simulink model "HVDCMMCInterconnection"  (R2023b)
settings: Solver=FixedStepDiscrete  StartTime=0.0  StopTime=10  FixedStep=Ts_Power  RelTol=1e-4
PreLoadFcn:
  | HVDCMMCInterconnectionParam
StartFcn:
  | tic
StopFcn:
  | toc
values from neighbouring files (symbols this model uses):
  C_PM = 1.758e-3    (= 0.001758)    [HVDCMMCInterconnectionParam.m]
  Cg = 50e-9    (= 5e-08)    [HVDCMMCInterconnectionParam.m]
  D_R = 0.001    [HVDCMMCInterconnectionParam.m]
  D_Rs = 1e8    (= 100000000)    [HVDCMMCInterconnectionParam.m]
  D_Vf = 0    [HVDCMMCInterconnectionParam.m]
  Fnom = 50    [HVDCMMCInterconnectionParam.m]
  HRM = 2    [HVDCMMCInterconnectionParam.m]
  Ki_Ireg = 6    [HVDCMMCInterconnectionParam.m]
  Ki_Preg = 1.0    (= 1)    [HVDCMMCInterconnectionParam.m]
  Ki_Qreg = 1.0    (= 1)    [HVDCMMCInterconnectionParam.m]
  Ki_VDCreg = 100    [HVDCMMCInterconnectionParam.m]
  Kp_Ireg = 0.6    [HVDCMMCInterconnectionParam.m]
  Kp_Preg = 0.5/3    (= 0.166666666667)    [HVDCMMCInterconnectionParam.m]
  Kp_Qreg = 0.5/3    (= 0.166666666667)    [HVDCMMCInterconnectionParam.m]
  Kp_VDCreg = 4    [HVDCMMCInterconnectionParam.m]
  L_cable = 15e-3    (= 0.015)    [HVDCMMCInterconnectionParam.m]
  Larm = Larm_pu*(Zb_ac/(2*pi*Fnom))    [HVDCMMCInterconnectionParam.m]
  Lff = Larm_pu/2    (= 0.075)    [HVDCMMCInterconnectionParam.m]
  Limits_Ireg = [ 2.0  -2.0]    [HVDCMMCInterconnectionParam.m]
  Limits_Preg = [ 1.2, 0.8 ]    [HVDCMMCInterconnectionParam.m]
  Limits_Qreg = [ 0.25, -0.25 ]    [HVDCMMCInterconnectionParam.m]
  Limits_VDCreg = [ 2.0  -2.0]    [HVDCMMCInterconnectionParam.m]
  Lxfo = 0.12    [HVDCMMCInterconnectionParam.m]
  Nb_PM = 36    [HVDCMMCInterconnectionParam.m]
  Pnom = 1000e6    (= 1000000000)    [HVDCMMCInterconnectionParam.m]
  R_cable = 0.5    [HVDCMMCInterconnectionParam.m]
  R_startup = 400    [HVDCMMCInterconnectionParam.m]
  Rarm = Rarm_pu*Zb_ac    [HVDCMMCInterconnectionParam.m]
  Rff = Rarm_pu/2    (= 0.00075)    [HVDCMMCInterconnectionParam.m]
  Rg = 100    [HVDCMMCInterconnectionParam.m]
  Rxfo = 0.003    [HVDCMMCInterconnectionParam.m]
  Slope_Pref = 0.5    [HVDCMMCInterconnectionParam.m]
  Slope_Qref = 0.5    [HVDCMMCInterconnectionParam.m]
  Slope_Vdc_ref = Vnom_dc/5    (= 128000)    [HVDCMMCInterconnectionParam.m]
  Tbrk1_On = 0.1    [HVDCMMCInterconnectionParam.m]
  Tbrk2_On = 1.0    (= 1)    [HVDCMMCInterconnectionParam.m]
  Tdeblock = 1.5    [HVDCMMCInterconnectionParam.m]
  Tfault = 9999    [HVDCMMCInterconnectionParam.m]
  Ton_Converter2 = 4    [HVDCMMCInterconnectionParam.m]
  Ton_PQreg = 4    [HVDCMMCInterconnectionParam.m]
  Ton_VDCreg = 1.5    [HVDCMMCInterconnectionParam.m]
  Ts = Ts_Control    (= 4e-05)    [HVDCMMCInterconnectionParam.m]    (also in power_circ2ss_sps_calc.m = 1e-06)
  Ts_Control = 40e-6    (= 4e-05)    [HVDCMMCInterconnectionParam.m]
  Ts_Power = 20e-6    (= 2e-05)    [HVDCMMCInterconnectionParam.m]
  Vb_ac = sqrt(2/3)*Vnom_sec    [HVDCMMCInterconnectionParam.m]
  Vb_dc = Vnom_dc    (= 640000)    [HVDCMMCInterconnectionParam.m]
  Vc0_PM = 0    [HVDCMMCInterconnectionParam.m]
  Vnom_dc = 640e3    (= 640000)    [HVDCMMCInterconnectionParam.m]
  Vnom_prim = 400e3    (= 400000)    [HVDCMMCInterconnectionParam.m]
  Vnom_sec = 333e3    (= 333000)    [HVDCMMCInterconnectionParam.m]
  w = 2*pi*Fnom    (= 314.159265359)    [HVDCMMCInterconnectionParam.m]
undefined symbols (not defined in the file or in its folder): ACDC, ACDC3, DiscIntNeverNeededParam, gcbh, Pcc, S, sps_AC, sps_rtmsupport
libraries: simulink x61, spsControlledVoltageSourceLib x56, spsCurrentMeasurementLib x56, spsDiodeLib x40, spsSeriesRLCBranchLib x32, spsVoltageMeasurementLib x20, powerlib_extras x9, spsHalfBridgeMMCmodel x8, spsGroundLib x7, spsSecondOrderFilterLib x6, spsabctodq0Lib x6, spsMeanLib x3
(part 1 of 11)
settings Model: SimulationMode=accelerator  Creator=The MathWorks, Inc.  LastModifiedBy=rober
settings SolverCC: ZeroCrossAlgorithm=Adaptive  InsertRTBMode=Always
settings DataIOCC: SaveFormat=StructureWithTime  SaveOutput=off  SignalLogging=off  DSMLogging=off  SaveTime=off  ReturnWorkspaceOutputs=off
settings OptimizationCC: ReuseModelBlockBuffer=off  ExpressionDepthLimit=2147483647  LifeSpan=inf
settings DebuggingCC: UnderspecifiedInitializationDetection=Classic  MergeDetectMultiDrivingBlocksExec=none  SolverPrmCheckMsg=warning  FcnCallInpInsideContextMsg=warning  AllowSymbolicDim=off  StateNameClashWarn=warning  SFUnexpectedBacktrackingDiag=warning  SFNoUnconditionalDefaultTransitionDiag=warning  SFExecutionAtInitializationDiag=none  ArithmeticOperatorsInVariantConditions=warning
settings HardwareCC: ProdBitPerPointer=32  ProdBitPerSizeT=32  ProdBitPerPtrDiffT=32  ProdLargestAtomicFloat=None  ProdIntDivRoundTo=Undefined  ProdEndianess=Unspecified  ProdWordSize=32  ProdHWDeviceType=32-bit Generic
settings ModelReferenceCC: EnableRefExpFcnMdlSchedulingChecks=on  EnableParallelModelReferenceBuilds=on  ModelReferenceMinAlgLoopOccurrences=on  PropagateSignalLabelsOutOfModel=off
settings SFSimCC: SimUseLocalCustomCode=off  CustomCodeUndefinedFunction=UseInterfaceOnly
settings RTWCC: RTWUseLocalCustomCode=off
settings CodeAppCC: StateflowObjectComments=on
settings GRTTargetCC: CombineOutputUpdateFcns=off  GRTInterface=on
settings ConfigComp: CovMetricSettings=dw  CovSaveCumulativeToWorkspaceVar=on  CovSaveSingleToWorkspaceVar=on  CovExternalEMLEnable=off
settings SimscapeCC: SimscapeNormalizeSystem=off

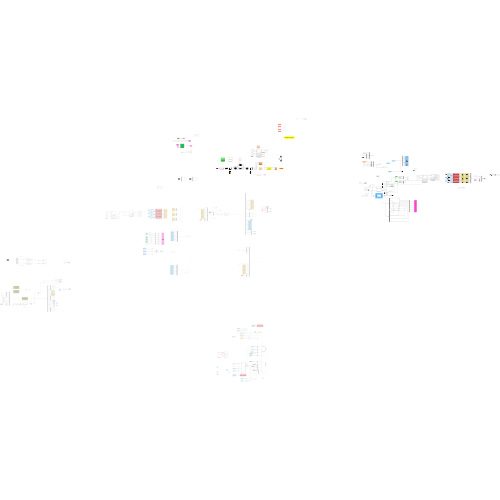
[thumbnail: Simulink's stored preview of the top-level diagram]
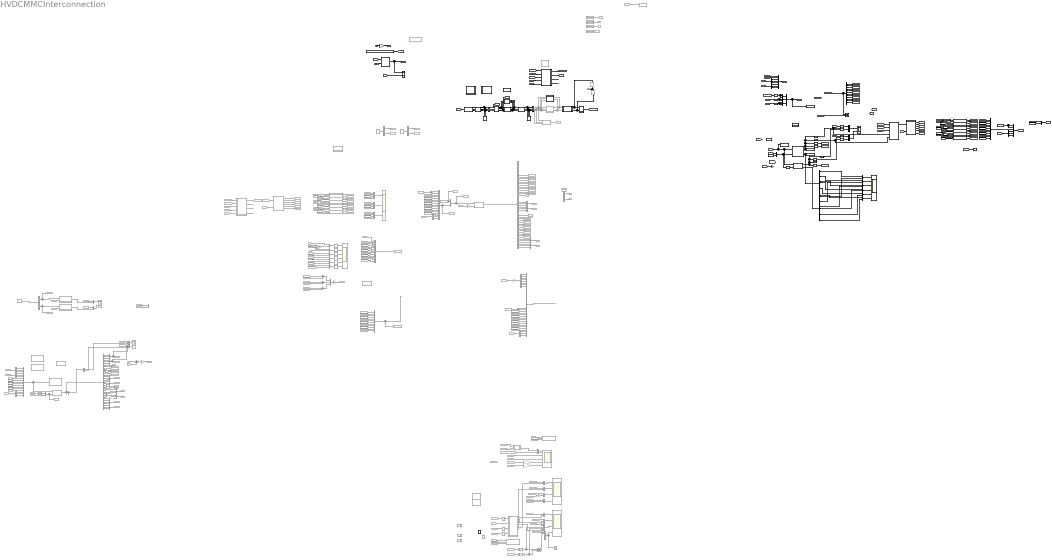
== system HVDCMMCInterconnection ==
  note: HVDC-MMC Control System
  3ph SM1 : Subsystem  Commented=on
  3ph SM10 : Subsystem
  3ph SM11 : Subsystem
  3ph SM12 : Subsystem
  3ph SM13 : Subsystem
  3ph SM14 : Subsystem
  3ph SM2 : Subsystem  Commented=on
  3ph SM3 : Subsystem  Commented=on
  3ph SM4 : Subsystem  Commented=on
  3ph SM5 : Subsystem  Commented=on
  3ph SM6 : Subsystem  Commented=on
  3ph SM7 : Subsystem  Commented=on
  3ph SM8 : Subsystem  Commented=on
  3ph SM9 : Subsystem
  Add1 : Sum  Commented=on  Inputs=-+
  BRK_CTRL : Subsystem  Commented=on
  BRK_CTRL1 : Subsystem  Commented=on
  Brk1 : spsThreePhaseBreakerLib/Three-Phase Breaker  InitialState=open  SwitchA=on  SwitchB=on  SwitchC=on  SwitchTimes=0.1  External=on  BreakerResistance=0.01  SnubberResistance=1e6  SnubberCapacitance=inf  Measurements=None
  Brk2 : spsThreePhaseBreakerLib/Three-Phase Breaker  InitialState=open  SwitchA=on  SwitchB=on  SwitchC=on  SwitchTimes=[30/60]*10000  External=on  BreakerResistance=0.01  SnubberResistance=1e6  SnubberCapacitance=inf  Measurements=None
  COMPARE1 : Scope  Commented=on  NumInputPorts=6
  COMPARE2 : Scope  NumInputPorts=6
  Cast To Double : DataTypeConversion  Commented=on  OutDataTypeStr=double  SaturateOnIntegerOverflow=off  RndMeth=Floor
  Cast To Double1 : DataTypeConversion  Commented=on  OutDataTypeStr=double  SaturateOnIntegerOverflow=off  RndMeth=Floor
  Cast To Double2 : DataTypeConversion  OutDataTypeStr=double  SaturateOnIntegerOverflow=off  RndMeth=Floor
  Cast To Double3 : DataTypeConversion  OutDataTypeStr=double  SaturateOnIntegerOverflow=off  RndMeth=Floor
  Cast To Double4 : DataTypeConversion  OutDataTypeStr=double  SaturateOnIntegerOverflow=off  RndMeth=Floor
  Clock : Clock
  Constant : Constant  Value=zeros(12,1)
  Constant1 : Constant  Commented=on  Value=Vnom_dc/2  SampleTime=Ts_Power
  Constant2 : Constant  Commented=on  Value=Vnom_dc/2  SampleTime=Ts_Power
  Constant3 : Constant  Value=complex( [[ 0 Vnom_prim*sqrt(2/3); 0 0; 0 0] zeros(3,HRM-1) ])
  Constant4 : Constant  Value=Vnom_dc/2  SampleTime=Ts_Power
  Control : Subsystem
  Control1 : Subsystem  Commented=on
  Control2 : Subsystem
  Conv 2 : Subsystem
      settings: PortSchema="{\"entries\":[{\"content\":{\"sides\":[{\"content\":{\"connectorIds\":[\"LConn1\",\"LConn2\"]},\"type\":\"ConnectorPlacement.EquallySpacedRectSide\",\"uuid\":\"34e68c3c-08e2-4036-96f4-bd6ca1a4adc7\"},{\"content\":{\"connectorIds\":[\"In1\"],\"side\":\"RIGHT\"},\"type\":\"ConnectorPlacement.EquallySpacedRectSide\",\"uuid\":\"8026f2da-b291-4e86-8efa-4dfa5391ad34\"},{\"content\":{\"side\":\"TOP\"},\"type\":\"ConnectorPlacement.EquallySpacedRectSide\",\"uuid\":\"2a5049d1-3deb-4ece-8237-adb3b31cd77f\"}]},\"type\":\"ConnectorPlacement.EquallySpacedConnector\",\"uuid\":\"95075630-e580-4539-9cf3-c9c75bab0a7f\"}],\"packageUris\":[\"http://schema.mathworks.com/mf0/Connector/R2020b\"],\"version\":\"1.0\"}"
  DC & converter 2 : Subsystem
      mask Display: disp('DC circuit')
  DQn->ABC : MATLAB Function  TreatAsAtomicUnit=on  SystemSampleTime=Ts_Power  mask{N=HRM}
      mask prompts: N "Harmonic order:"
  DSS : Subsystem  Commented=on  SystemSampleTime=Ts_Power  mask{A=ACDC3.A, B=ACDC3.B, C=ACDC3.C, D=ACDC3.D, InitVec=ACDC3.x0, dt=Ts_Power, DQSYM=off, N=HRM, Ws=w}
      mask prompts: InitVec "Initial condition:"; dt "Time step (s):"; N "Harmonic number:"; Ws "Angular frequency (1/rad):"
      mask init:
      | % I = eye(size(A,1));
      | % INVR = I/(I-A*dt/2);
      | % Ad1 = INVR*(I+A*dt/2);
      | % Bd1 = INVR*B*dt/2;
      | % Cd1 = C*Ad1;
      | % Dd11 = C*INVR*B*dt/2+D;
      | % Dd12 = C*INVR*B*dt/2;
      | 
      |     I = eye(size(A,1));
      |     INVR = I/(I-A*dt/2);
      |     Ad1 = INVR*(I+A*dt/2);
      |     Bd1 = INVR*B;
      |     Cd1 = C*INVR*dt;
      |     Dd1 = Cd1*B/2 + D;
      | 
      | DQSYM = get_param(gcb,'DQSYM');
      | 
      | comp = 0;
      | 
      | if(strcmp(DQSYM,'on'))
      | 
      | %Calculating the PNZ matrices
      | 
      |     a = -0.5+0.866i;
      |     a2 = -0.5-0.866i;
      |     Sas = [1,a,a2;1,a2,a;1,1,1]/3;
      | 
      |     arows = size(Ad1,1)/3; %signal size
      |     acols = size(Ad1,2)/3; %signal size
      | 
      |     brows = size(Bd1,1)/3; %signal size
      |     bcols = size(Bd1,2)/3; %signal size
      | 
      |     crows = size(Cd1,1)/3; %signal size
      |     ccols = size(Cd1,2)/3; %signal size
      | 
      |     d1rows = size(Dd1,1)/3; %signal size
      |     d1cols = size(Dd1,2)/3; %signal size
      | 
      |     %%%%%%%%%%%%%%%%%%%%%%% Check for inconsistencies  %%%%%%%%%%%%%%%%%%%%%%%
      | 
      |     szMatA = size(A,1);
      |     iL = eye(szMatA);
      |     szMatiL = size(iL,1);
      | 
      |     if(szMatiL ~= szMatA || size(A,1) ~= size(A,2) || size(iL,1) ~= size(iL,2))
      |         error('[Int_DQN_Mat/swFeedback] check matrix A size!');
      |     end
      | 
      |     if(arows ~= brows || acols ~= ccols || crows ~= d1rows || bcols ~= d1cols)
      |         error('[Int_DQN_Mat/Initialize] the sizes of the state-space matrices!');
      |     end
      | 
      |     %%%%%%%%%%%%%%%%%%%%%%%%%%%%%%%%%%%%%%%%%%%%%%%%%%%%%%%%%%%%%%%
      | 
      | 
      |     %%%%%%%%%%%%%%%%%%%%%%% A --> Bpnz %%%%%%%%%%%%%%%%%%%%%%%
      |     Adc = complex(zeros(3*arows,3*acols));
      | 
      |     for i = 1 : arows
      |         for j = 1 : acols
      |             Adc((1:3) + (i-1)*3,(1:3) + (j-1)*3) = Sas*Ad1((1:3) + (i-1)*3,(1:3) + (j-1)*3)/Sas;
      |             %Adc((1:3) + (i-1)*3,(1:3) + (j-1)*3) = diag(diag(real(Adc((1:3) + (i-1)*3,(1:3) + (j-1)*3))));
      |             %Adc((1:3) + (i-1)*3,(1:3) + (j-1)*3) = diag(diag((Adc((1:3) + (i-1)*3,(1:3) + (j-1)*3))));
      | 
      |         end
      |     end
      |     %%%%%%%%%%%%%%%%%%%%%%%%%%%%%%%%%%%%%%%%%%%%%%%%%%%%%%%%%%%%%%%
      | 
      |     %%%%%%%%%%%%%%%%%%%%%%% B --> Bpnz %%%%%%%%%%%%%%%%%%%%%%%
      | 
      |     Bdc = complex(zeros(3*brows,3*bcols));
      | 
      |     for i = 1 : brows
      |         for j = 1 : bcols
      |             Bdc((1:3) + (i-1)*3,(1:3) + (j-1)*3) = Sas*Bd1((1:3) + (i-1)*3,(1:3) + (j-1)*3)/Sas;
      |             %Bdc((1:3) + (i-1)*3,(1:3) + (j-1)*3) = diag(diag(real(Bdc((1:3) + (i-1)*3,(1:3) + (j-1)*3))));
      |             %Bdc((1:3) + (i-1)*3,(1:3) + (j-1)*3) = diag(diag((Bdc((1:3) + (i-1)*3,(1:3) + (j-1)*3))));
      | 
      |         end
      |     end
      |     %%%%%%%%%%%%%%%%%%%%%%%%%%%%%%%%%%%%%%%%%%%%%%%%%%%%%%%%%%%%%%%
      | 
      |     %%%%%%%%%%%%%%%%%%%%%%% C --> Cpnz %%%%%%%%%%%%%%%%%%%%%%%
      | 
      |     Cdc = complex(zeros(3*crows,3*ccols));
      | 
      |     for i = 1 : crows
      |         for j = 1 : ccols
      |             Cdc((1:3) + (i-1)*3,(1:3) + (j-1)*3) = Sas*Cd1((1:3) + (i-1)*3,(1:3) + (j-1)*3)/Sas;
      |             %Cdc((1:3) + (i-1)*3,(1:3) + (j-1)*3) = diag(diag(real(Cdc((1:3) + (i-1)*3,(1:3) + (j-1)*3))));
      |             %Cdc((1:3) + (i-1)*3,(1:3) + (j-1)*3) = diag(diag((Cdc((1:3) + (i-1)*3,(1:3) + (j-1)*3))));
      |         end
      |     end
      |     %%%%%%%%%%%%%%%%%%%%%%%%%%%%%%%%%%%%%%%%%%%%%%%%%%%%%%%%%%%%%%%
      | 
      |     
      |     %%%%%%%%%%%%%%%%%%%%%%% D1 --> Cpnz %%%%%%%%%%%%%%%%%%%%%%%
      | 
      |     Ddc = complex(zeros(3*d1rows,3*d1cols));
      | 
      |     for i = 1 : d1rows
      |         for j = 1 : d1cols
      |             Ddc((1:3) + (i-1)*3,(1:3) + (j-1)*3) = Sas*Dd1((1:3) + (i-1)*3,(1:3) + (j-1)*3)/Sas;
      |             %Ddc1((1:3) + (i-1)*3,(1:3) + (j-1)*3) = diag(diag(real(Ddc1((1:3) + (i-1)*3,(1:3) + (j-1)*3))));
      |             %Ddc((1:3) + (i-1)*3,(1:3) + (j-1)*3) = diag(diag((Ddc((1:3) + (i-1)*3,(1:3) + (j-1)*3))));
      |         end
      |     end
      |     %%%%%%%%%%%%%%%%%%%%%%%%%%%%%%%%%%%%%%%%%%%%%%%%%%%%%%%%%%%%%%%
      | 
      |     Adc(abs(Adc)<2*eps) = 0;
      |     Bdc(abs(Bdc)<2*eps) = 0;
      |     Cdc(abs(Cdc)<2*eps) = 0;
      |     Ddc(abs(Ddc)<2*eps) = 0;
      | 
      |     InitVec_c = complex(zeros(brows*3,N+1));
      | 
      | 
      |     if(~isempty(InitVec))
      |         if(mod(numel(InitVec),3)~=0) 
      |             warning('[SS_DQNc_Mat] InitVec with wrong size --> needs to be a multiple of 3!'); 
      | 
      |         else
      |             for k = 1 : numel(InitVec)/3
      |                 InitVec_c((k-1)*3+1:(k-1)*3+3,1) = Sas*InitVec((k-1)*3+1:(k-1)*3+3)*exp(+1i*Ws*dt);
      |             end
      |         end
      |     end
      | 
      |     InitVec = InitVec_c;
      | 
      | 
      |     Ad1 = Adc;
      |     Bd1 = Bdc;
      |     Cd1 = Cdc;
      |     Dd1 = Ddc;
      | 
      |     comp = -1i*Ws*dt;
      | 
      | end
      settings: MinAlgLoopOccurrences=on
      settings: LibrarySourceBlock=|
      | spsSynchronousMachineModel/Discrete robust/State Space Model/Discretize
      | BE or Tustin
      mask Callback DQSYM:
      | EMT = get_param(gcb,'DQSYM');
      | 
      | if(strcmp(EMT,'on'))
      |    set_param(gcb,'MaskVisibilities',{'on','on','on','on','on','on','on','on','on'});
      | else
      |    set_param(gcb,'MaskVisibilities',{'on','on','on','on','on','on','on','off','off'});
      | end
      mask Display: disp(['{\color{red}\bf\fontsize{12}x(t) = Ad*x(t-dt)+Bd*u(t)}',newline,'{\color{gray}\bf\fontsize{12}y(t) = Cd*x(t-dt)+Dd*u(t)}'], 'texmode','on');
  DSS1 : Subsystem  Commented=on  SystemSampleTime=Ts_Power  mask{A=ACDC3.A, B=ACDC3.B, C=ACDC3.C, D=ACDC3.D, InitVec=ACDC3.x0, dt=Ts_Power, NrBrk=6, DQSYM=off, N=HRM, Ws=w}
      mask prompts: InitVec "Initial condition:"; dt "Time step (s):"; NrBrk "Number of breakers:"; N "Harmonic number:"; Ws "Angular frequency (1/rad):"
      mask init:
      | % I = eye(size(A,1));
      | % INVR = I/(I-A*dt/2);
      | % Ad1 = INVR*(I+A*dt/2);
      | % Bd1 = INVR*B*dt/2;
      | % Cd1 = C*Ad1;
      | % Dd11 = C*INVR*B*dt/2+D;
      | % Dd12 = C*INVR*B*dt/2;
      | 
      |     I = eye(size(A,1));
      |     INVR = I/(I-A*dt/2);
      |     Ad1 = INVR*(I+A*dt/2);
      |     Bd1 = INVR*B;
      |     Cd1 = C*INVR*dt;
      |     Dd1 = Cd1*B/2 + D;
      | 
      | DQSYM = get_param(gcb,'DQSYM');
      | 
      | comp = 0;
      | 
      |     arows = size(Ad1,1)/3; %signal size
      |     acols = size(Ad1,2)/3; %signal size
      | 
      |     brows = size(Bd1,1)/3; %signal size
      |     bcols = size(Bd1,2)/3; %signal size
      | 
      |     crows = size(Cd1,1)/3; %signal size
      |     ccols = size(Cd1,2)/3; %signal size
      | 
      |     d1rows = size(Dd1,1)/3; %signal size
      |     d1cols = size(Dd1,2)/3; %signal size
      | 
      | if(strcmp(DQSYM,'on'))
      | 
      | %Calculating the PNZ matrices
      | 
      |     a = -0.5+0.866i;
      |     a2 = -0.5-0.866i;
      |     Sas = [1,a,a2;1,a2,a;1,1,1]/3;
      | 
      | 
      | 
      |     %%%%%%%%%%%%%%%%%%%%%%% Check for inconsistencies  %%%%%%%%%%%%%%%%%%%%%%%
      | 
      |     szMatA = size(A,1);
      |     iL = eye(szMatA);
      |     szMatiL = size(iL,1);
      | 
      |     if(szMatiL ~= szMatA || size(A,1) ~= size(A,2) || size(iL,1) ~= size(iL,2))
      |         error('[Int_DQN_Mat/swFeedback] check matrix A size!');
      |     end
      | 
      |     if(arows ~= brows || acols ~= ccols || crows ~= d1rows || bcols ~= d1cols)
      |         error('[Int_DQN_Mat/Initialize] the sizes of the state-space matrices!');
      |     end
      | 
      |     %%%%%%%%%%%%%%%%%%%%%%%%%%%%%%%%%%%%%%%%%%%%%%%%%%%%%%%%%%%%%%%
      | 
      | 
      |     %%%%%%%%%%%%%%%%%%%%%%% A --> Bpnz %%%%%%%%%%%%%%%%%%%%%%%
      |     Adc = complex(zeros(3*arows,3*acols));
      | 
      |     for i = 1 : arows
      |         for j = 1 : acols
      |             Adc((1:3) + (i-1)*3,(1:3) + (j-1)*3) = Sas*Ad1((1:3) + (i-1)*3,(1:3) + (j-1)*3)/Sas;
      |             %Adc((1:3) + (i-1)*3,(1:3) + (j-1)*3) = diag(diag(real(Adc((1:3) + (i-1)*3,(1:3) + (j-1)*3))));
      |             %Adc((1:3) + (i-1)*3,(1:3) + (j-1)*3) = diag(diag((Adc((1:3) + (i-1)*3,(1:3) + (j-1)*3))));
      | 
      |         end
      |     end
      |     %%%%%%%%%%%%%%%%%%%%%%%%%%%%%%%%%%%%%%%%%%%%%%%%%%%%%%%%%%%%%%%
      | 
      |     %%%%%%%%%%%%%%%%%%%%%%% B --> Bpnz %%%%%%%%%%%%%%%%%%%%%%%
      | 
      |     Bdc = complex(zeros(3*brows,3*bcols));
      | 
      |     for i = 1 : brows
      |         for j = 1 : bcols
      |             Bdc((1:3) + (i-1)*3,(1:3) + (j-1)*3) = Sas*Bd1((1:3) + (i-1)*3,(1:3) + (j-1)*3)/Sas;
      |             %Bdc((1:3) + (i-1)*3,(1:3) + (j-1)*3) = diag(diag(real(Bdc((1:3) + (i-1)*3,(1:3) + (j-1)*3))));
      |             %Bdc((1:3) + (i-1)*3,(1:3) + (j-1)*3) = diag(diag((Bdc((1:3) + (i-1)*3,(1:3) + (j-1)*3))));
      | 
      |         end
      |     end
      |     %%%%%%%%%%%%%%%%%%%%%%%%%%%%%%%%%%%%%%%%%%%%%%%%%%%%%%%%%%%%%%%
      | 
      |     %%%%%%%%%%%%%%%%%%%%%%% C --> Cpnz %%%%%%%%%%%%%%%%%%%%%%%
      | 
      |     Cdc = complex(zeros(3*crows,3*ccols));
      | 
      |     for i = 1 : crows
      |         for j = 1 : ccols
      |             Cdc((1:3) + (i-1)*3,(1:3) + (j-1)*3) = Sas*Cd1((1:3) + (i-1)*3,(1:3) + (j-1)*3)/Sas;
      |             %Cdc((1:3) + (i-1)*3,(1:3) + (j-1)*3) = diag(diag(real(Cdc((1:3) + (i-1)*3,(1:3) + (j-1)*3))));
      |             %Cdc((1:3) + (i-1)*3,(1:3) + (j-1)*3) = diag(diag((Cdc((1:3) + (i-1)*3,(1:3) + (j-1)*3))));
      |         end
      |     end
      |     %%%%%%%%%%%%%%%%%%%%%%%%%%%%%%%%%%%%%%%%%%%%%%%%%%%%%%%%%%%%%%%
      | 
      |     
      |     %%%%%%%%%%%%%%%%%%%%%%% D1 --> Cpnz %%%%%%%%%%%%%%%%%%%%%%%
      | 
      |     Ddc = complex(zeros(3*d1rows,3*d1cols));
      | 
      |     for i = 1 : d1rows
      |         for j = 1 : d1cols
      |             Ddc((1:3) + (i-1)*3,(1:3) + (j-1)*3) = Sas*Dd1((1:3) + (i-1)*3,(1:3) + (j-1)*3)/Sas;
      |             %Ddc1((1:3) + (i-1)*3,(1:3) + (j-1)*3) = diag(diag(real(Ddc1((1:3) + (i-1)*3,(1:3) + (j-1)*3))));
      |             %Ddc((1:3) + (i-1)*3,(1:3) + (j-1)*3) = diag(diag((Ddc((1:3) + (i-1)*3,(1:3) + (j-1)*3))));
      |         end
      |     end
      |     %%%%%%%%%%%%%%%%%%%%%%%%%%%%%%%%%%%%%%%%%%%%%%%%%%%%%%%%%%%%%%%
      | 
      |     Adc(abs(Adc)<2*eps) = 0;
      |     Bdc(abs(Bdc)<2*eps) = 0;
      |     Cdc(abs(Cdc)<2*eps) = 0;
      |     Ddc(abs(Ddc)<2*eps) = 0;
      | 
      |     InitVec_c = complex(zeros(brows*3,N+1));
      | 
      | 
      |     if(~isempty(InitVec))
      |         if(mod(numel(InitVec),3)~=0) 
      |             warning('[SS_DQNc_Mat] InitVec with wrong size --> needs to be a multiple of 3!'); 
      | 
      |         else
      |             for k = 1 : numel(InitVec)/3
      |                 InitVec_c((k-1)*3+1:(k-1)*3+3,1) = Sas*InitVec((k-1)*3+1:(k-1)*3+3)*exp(+1i*Ws*dt);
      |             end
      |         end
      |     end
      | 
      |     InitVec = InitVec_c;
      | 
      | 
      |     Ad1 = Adc;
      |     Bd1 = Bdc;
      |     Cd1 = Cdc;
      |     Dd1 = Ddc;
      | 
      |     comp = -1i*Ws*dt;
      | 
      | 
      | end
      | 
      |     
      |     Ad11 = Ad1(1:NrBrk,1:NrBrk);        if(isempty(Ad11)) Ad11 = zeros(3,3); end
      |     Ad12 = Ad1(1:NrBrk,NrBrk+1:end);    if(isempty(Ad12)) Ad12 = zeros(3,3); end
      |     Ad21 = Ad1(NrBrk+1:end,1:NrBrk);    if(isempty(Ad21)) Ad21 = zeros(3,3); end
      |     Ad22 = Ad1(NrBrk+1:end,NrBrk+1:end); if(isempty(Ad22)) Ad22 = zeros(3,3); end
      | 
      |     Bd11 = Bd1(1:NrBrk,1:NrBrk);        if(isempty(Bd11)) Bd11 = zeros(3,3); end
      |     Bd12 = Bd1(1:NrBrk,NrBrk+1:end);    if(isempty(Bd12)) Bd12 = zeros(3,3); end
      |     Bd21 = Bd1(NrBrk+1:end,1:NrBrk);    if(isempty(Bd21)) Bd21 = zeros(3,3); end
      |     Bd22 = Bd1(NrBrk+1:end,NrBrk+1:end); if(isempty(Bd22)) Bd22 = zeros(3,3*bcols-NrBrk); end
      | 
      |     Cd11 = Cd1(1:NrBrk,1:NrBrk);        if(isempty(Cd11)) Cd11 = zeros(3,3); end
      |     Cd12 = Cd1(1:NrBrk,NrBrk+1:end);    if(isempty(Cd12)) Cd12 = zeros(3,3); end
      |     Cd21 = Cd1(NrBrk+1:end,1:NrBrk);    if(isempty(Cd21)) Cd21 = zeros(3,3); end
      |     Cd22 = Cd1(NrBrk+1:end,NrBrk+1:end); if(isempty(Cd22)) Cd22 = zeros(3*crows-NrBrk,3*ccols); end
      | 
      |     Dd11 = Dd1(1:NrBrk,1:NrBrk);        if(isempty(Dd11)) Dd11 = zeros(3,3); end
      |     Dd12 = Dd1(1:NrBrk,NrBrk+1:end);    if(isempty(Dd12)) Dd12 = zeros(3,3); end
      |     Dd21 = Dd1(NrBrk+1:end,1:NrBrk);    if(isempty(Dd21)) Dd21 = zeros(3,3); end
      |     Dd22 = Dd1(NrBrk+1:end,NrBrk+1:end); if(isempty(Dd22)) Dd22 = zeros(3,3); end
      | 
      | 
      | 
      | 
      | InitVecS = InitVec(1:NrBrk);
      | 
      | InitVecNS = InitVec(NrBrk+1:end); if(isempty(InitVecNS)) InitVecNS = 0; end
      settings: MinAlgLoopOccurrences=on
      settings: LibrarySourceBlock=|
      | spsSynchronousMachineModel/Discrete robust/State Space Model/Discretize
      | BE or Tustin
      mask Display: disp(['{\color{red}\bf\fontsize{12}x(t) = Ad*x(t-dt)+Bd*u(t)}',newline,'{\color{gray}\bf\fontsize{12}y(t) = Cd*x(t-dt)+Dd*u(t)}'], 'texmode','on');
  DSS2 : Subsystem  Commented=on  SystemSampleTime=Ts_Power  mask{A=ACDC3.A, B=ACDC3.B, C=ACDC3.C, D=ACDC3.D, InitVec=ACDC3.x0, dt=Ts_Power, NrBrk=6, DQSYM=off, N=HRM, Ws=w}
      mask prompts: InitVec "Initial condition:"; dt "Time step (s):"; NrBrk "Number of breakers:"; N "Harmonic number:"; Ws "Angular frequency (1/rad):"
      mask init: same as HVDCMMCInterconnection/DSS1
      settings: MinAlgLoopOccurrences=on
      settings: LibrarySourceBlock=|
      | spsSynchronousMachineModel/Discrete robust/State Space Model/Discretize
      | BE or Tustin
      mask Display: disp(['{\color{red}\bf\fontsize{12}x(t) = Ad*x(t-dt)+Bd*u(t)}',newline,'{\color{gray}\bf\fontsize{12}y(t) = Cd*x(t-dt)+Dd*u(t)}'], 'texmode','on');
  Delay{,3,10..11} (4 alike) : Delay  Commented=on  DelayLength=1  SampleTime=Ts_Power
  Delay2 : Delay  DelayLength=1  SampleTime=Ts_Power
  Delay5 : Subsystem  Commented=on
  Delay6 : Subsystem  Commented=on
  Delay7 : Subsystem  Commented=on
  Delay8 : Subsystem  Commented=on
  Delay9 : Subsystem  Commented=on
  Demux{,4..5,8} (4 alike) : Demux  Commented=on  Outputs=2
  Demux{1..3,12,14} (5 alike) : Demux  Commented=on  Outputs=3
  Demux10 : Demux  Outputs=3
  Demux11 : Demux  Outputs=3
  Demux13 : Demux  Commented=on  Outputs=8
  Demux15 : Demux  Outputs=20
  Demux16 : Demux  Outputs=20
  Demux17 : Demux  Outputs=12
  Demux18 : Demux  Outputs=3
  Demux6 : Demux  Commented=on  Outputs=numel(ACDC3.outputs)
  Demux7 : Demux  Commented=on  Outputs=[6,27]
  Demux9 : Demux  Commented=on  Outputs=numel(ACDC.outputs)
  Discrete State-Space : DiscreteStateSpace  Commented=on  A=ACDC3.Adiscrete  B=ACDC3.Bdiscrete  C=ACDC3.Cdiscrete  D=ACDC3.Ddiscrete  InitialCondition=ACDC3.x0  SampleTime=Ts_Power
  Discrete State-Space1 : DiscreteStateSpace  Commented=on  A=ACDC.Adiscrete  B=ACDC.Bdiscrete  C=ACDC.Cdiscrete  D=ACDC.Ddiscrete  InitialCondition=ACDC.x0  SampleTime=Ts_Power
  From : From  Commented=on  GotoTag=Uref_Ap  TagVisibility=global
  From1 : From  Commented=on  GotoTag=Uref_An  TagVisibility=global
  From10 : From  Commented=on  GotoTag=IBrk2_EMT  TagVisibility=global
  From100 : From  Commented=on  GotoTag=PQreg_On  TagVisibility=global
  From102 : From  Commented=on  GotoTag=Ap_Vin  TagVisibility=global
  From103 : From  Commented=on  GotoTag=Ap_Vbl  TagVisibility=global
  From104 : From  Commented=on  GotoTag=Vdc_ref  TagVisibility=global
  From105 : From  Commented=on  GotoTag=Qref  TagVisibility=global
  From106 : From  Commented=on  GotoTag=Isec_ss
  From107 : From  Commented=on  GotoTag=I_Ap_Db  TagVisibility=global
  From108 : From  Commented=on  GotoTag=Uref_Ap_ss  TagVisibility=global
  From109 : From  Commented=on  GotoTag=Bp_Ipos
  From11 : From  Commented=on  GotoTag=Q
  From{36..37,91,110,117,120} (6 alike) : From  Commented=on  GotoTag=Ap_Ipos
  From111 : From  Commented=on  GotoTag=Cp_Ipos
  From112 : From  Commented=on  GotoTag=An_Ipos
  From{27,44,48,113} (4 alike) : From  Commented=on  GotoTag=I_Ap_Dt  TagVisibility=global
  From114 : From  Commented=on  GotoTag=Vdc2t  TagVisibility=global
  From115 : From  Commented=on  GotoTag=Vdc2b  TagVisibility=global
  From116 : From  Commented=on  GotoTag=Vsrc_ABC  TagVisibility=global
  From118 : From  Commented=on  GotoTag=I_Ap_Db  TagVisibility=global
  From{85,90,119,123} (4 alike) : From  Commented=on  GotoTag=Ap_Icap
  From12 : From  Commented=on  GotoTag=V12_Ap  TagVisibility=global
  From121 : From  Commented=on  GotoTag=Bn_Ipos
  From122 : From  Commented=on  GotoTag=Cn_Ipos
  From124 : From  Commented=on  GotoTag=Uref_Bn_ss  TagVisibility=global
  From125 : From  Commented=on  GotoTag=Bn_Ipos
  From126 : From  Commented=on  GotoTag=Bn_Icap
  From127 : From  Commented=on  GotoTag=Uref_Bp_ss  TagVisibility=global
  From128 : From  Commented=on  GotoTag=Bp_Ipos
  From129 : From  Commented=on  GotoTag=Bp_Icap
  From13 : From  Commented=on  GotoTag=V12_Am  TagVisibility=global
  From130 : From  Commented=on  GotoTag=Uref_Cn_ss  TagVisibility=global
  From131 : From  Commented=on  GotoTag=Cn_Ipos
  From132 : From  Commented=on  GotoTag=Cn_Icap
  From133 : From  Commented=on  GotoTag=Uref_Cp_ss  TagVisibility=global
  From134 : From  Commented=on  GotoTag=Cp_Ipos
  From135 : From  Commented=on  GotoTag=Cp_Icap
  From136 : From  Commented=on  GotoTag=Bn_Vin_EMT  TagVisibility=global
  From137 : From  Commented=on  GotoTag=Bn_Vbl_EMT  TagVisibility=global
  From138 : From  Commented=on  GotoTag=Bn_Vbl_ss
  From139 : From  Commented=on  GotoTag=Bn_Vin_ss
  From14 : From  Commented=on  GotoTag=V12_Bp  TagVisibility=global
  From140 : From  Commented=on  GotoTag=Cn_Vin_EMT  TagVisibility=global
  From141 : From  Commented=on  GotoTag=Cn_Vbl_EMT  TagVisibility=global
  From142 : From  Commented=on  GotoTag=Cn_Vbl_ss
  From143 : From  Commented=on  GotoTag=Cn_Vin_ss
  From144 : From  Commented=on  GotoTag=Vsrc_ABC  TagVisibility=global
  From145 : From  Commented=on  GotoTag=An_Vin_EMT  TagVisibility=global
  From146 : From  Commented=on  GotoTag=An_Vbl_EMT  TagVisibility=global
  From147 : From  Commented=on  GotoTag=Bn_Vin_EMT  TagVisibility=global
  From148 : From  Commented=on  GotoTag=Bn_Vbl_EMT  TagVisibility=global
  From149 : From  Commented=on  GotoTag=Bp_Vin_EMT  TagVisibility=global
  From15 : From  Commented=on  GotoTag=V12_Bm  TagVisibility=global
  From150 : From  Commented=on  GotoTag=Bp_Vbl_EMT  TagVisibility=global
  From151 : From  Commented=on  GotoTag=Ap_Vin_EMT  TagVisibility=global
  From152 : From  Commented=on  GotoTag=Ap_Vbl_EMT  TagVisibility=global
  From153 : From  Commented=on  GotoTag=Cn_Vin_EMT  TagVisibility=global
  From154 : From  Commented=on  GotoTag=Cn_Vbl_EMT  TagVisibility=global
  From155 : From  Commented=on  GotoTag=Cp_Vin_EMT  TagVisibility=global
  From156 : From  Commented=on  GotoTag=Cp_Vbl_EMT  TagVisibility=global
  From16 : From  Commented=on  GotoTag=V12_Cp  TagVisibility=global
  From164 : From  Commented=on  GotoTag=An_Vin_EMT  TagVisibility=global
  From165 : From  Commented=on  GotoTag=An_Vbl_EMT  TagVisibility=global
  From166 : From  Commented=on  GotoTag=Bn_Vin_EMT  TagVisibility=global
  From167 : From  Commented=on  GotoTag=Bn_Vbl_EMT  TagVisibility=global
  From168 : From  Commented=on  GotoTag=Bp_Vin_EMT  TagVisibility=global
  From169 : From  Commented=on  GotoTag=Bp_Vbl_EMT  TagVisibility=global
  From17 : From  Commented=on  GotoTag=V12_Cm  TagVisibility=global
  From174 : From  Commented=on  GotoTag=Ap_Vin_EMT  TagVisibility=global
  From175 : From  Commented=on  GotoTag=Ap_Vbl_EMT  TagVisibility=global
  From178 : From  Commented=on  GotoTag=Cn_Vin_EMT  TagVisibility=global
  From179 : From  Commented=on  GotoTag=Cn_Vbl_EMT  TagVisibility=global
  From18 : From  Commented=on  GotoTag=Vsrc_ABC  TagVisibility=global
  From180 : From  Commented=on  GotoTag=Cp_Vin_EMT  TagVisibility=global
  From181 : From  Commented=on  GotoTag=Cp_Vbl_EMT  TagVisibility=global
  From19 : From  Commented=on  GotoTag=Brk2_On  TagVisibility=global
  From198 : From  Commented=on  GotoTag=Id_ss
  From199 : From  Commented=on  GotoTag=Vsec_ss
  From2 : From  Commented=on  GotoTag=P
  From20 : From  Commented=on  GotoTag=Ip_ss
  From200 : From  Commented=on  GotoTag=Id_abc  TagVisibility=global
  From201 : From  Commented=on  GotoTag=Idc1p_ss
  From202 : From  Commented=on  GotoTag=Idc1n_ss
  From203 : From  Commented=on  GotoTag=Idc1  TagVisibility=global
  From204 : From  Commented=on  GotoTag=Vsec  TagVisibility=global
  From206 : From  Commented=on  GotoTag=Isec_ss
  From207 : From  Commented=on  GotoTag=Vdc_ss
  From208 : From  Commented=on  GotoTag=Vdc1  TagVisibility=global
  From209 : From  Commented=on  GotoTag=Uref_ABC  TagVisibility=global
  From210 : From  Commented=on  GotoTag=Uref_ABC_ss
  From22 : From  Commented=on  GotoTag=In_ss
  From24 : From  Commented=on  GotoTag=Brk1_On  TagVisibility=global
  From25 : From  Commented=on  GotoTag=Brk1_On  TagVisibility=global
  From26 : From  Commented=on  GotoTag=UBrk1_ss
  From28 : From  Commented=on  GotoTag=U_Ap_Dt
  From29 : From  Commented=on  GotoTag=Brk2_On  TagVisibility=global
  From30 : From  Commented=on  GotoTag=IBrk2_EMT  TagVisibility=global
  From31 : From  Commented=on  GotoTag=IBrk1_EMT  TagVisibility=global
  From33 : From  Commented=on  GotoTag=UBrk2_ss
  From34 : From  Commented=on  GotoTag=Uref_Ap  TagVisibility=global
  From35 : From  Commented=on  GotoTag=UBrk1_EMT  TagVisibility=global
  From39 : From  Commented=on  GotoTag=U_Ap_Dt
  From4 : From  Commented=on  GotoTag=Vdc_kV
  From40 : From  Commented=on  GotoTag=UBrk2_EMT  TagVisibility=global
  From47 : From  Commented=on  GotoTag=Uref_An_ss  TagVisibility=global
  From49 : From  Commented=on  GotoTag=An_Ipos
  From5 : From  Commented=on  GotoTag=V1rmsLL
  From51 : From  Commented=on  GotoTag=An_Icap
  From53 : From  Commented=on  GotoTag=Vsec_ss
  From54 : From  Commented=on  GotoTag=An_Vin_EMT  TagVisibility=global
  From55 : From  Commented=on  GotoTag=An_Vbl_EMT  TagVisibility=global
  From56 : From  Commented=on  GotoTag=IBRK
  From6 : From  Commented=on  GotoTag=Vsec_ABC
  From63 : From  Commented=on  GotoTag=BrkVec
  From64 : From  Commented=on  GotoTag=An_Vbl_ss
  From65 : From  Commented=on  GotoTag=Ig_abc  TagVisibility=global
  From66 : From  Commented=on  GotoTag=An_Vin_ss
  From67 : From  Commented=on  GotoTag=I_An_Db_EMT  TagVisibility=global
  From68 : From  Commented=on  GotoTag=I_An_Dt_EMT  TagVisibility=global
  From69 : From  Commented=on  GotoTag=U_Ap_SM
  From7 : From  Commented=on  GotoTag=An_Ipos
  From70 : From  Commented=on  GotoTag=I_Bn_Db_EMT  TagVisibility=global
  From71 : From  Commented=on  GotoTag=I_Bn_Dt_EMT  TagVisibility=global
  From72 : From  Commented=on  GotoTag=I_Bp_Db_EMT  TagVisibility=global
  From73 : From  Commented=on  GotoTag=I_Bp_Dt_EMT  TagVisibility=global
  From74 : From  Commented=on  GotoTag=I_Cn_Db_EMT  TagVisibility=global
  From75 : From  Commented=on  GotoTag=Uref_ABC_ss
  From76 : From  Commented=on  GotoTag=Blk  TagVisibility=global
  From77 : From  Commented=on  GotoTag=I_Cn_Dt_EMT  TagVisibility=global
  From78 : From  Commented=on  GotoTag=I_Cp_Db_EMT  TagVisibility=global
  From79 : From  Commented=on  GotoTag=I_Cp_Dt_EMT  TagVisibility=global
  From8 : From  Commented=on  GotoTag=IBrk1_EMT  TagVisibility=global
  From80 : From  Commented=on  GotoTag=I_Ap_Db_EMT  TagVisibility=global
  From81 : From  Commented=on  GotoTag=I_Ap_Dt_EMT  TagVisibility=global
  From82 : From  Commented=on  GotoTag=I_An_Db_EMT  TagVisibility=global
  From83 : From  Commented=on  GotoTag=I_An_Dt_EMT  TagVisibility=global
  From84 : From  Commented=on  GotoTag=I_Bn_Db_EMT  TagVisibility=global
  From86 : From  Commented=on  GotoTag=I_Bn_Dt_EMT  TagVisibility=global
  From87 : From  Commented=on  GotoTag=I_Bp_Db_EMT  TagVisibility=global
  From88 : From  Commented=on  GotoTag=I_Bp_Dt_EMT  TagVisibility=global
  From89 : From  Commented=on  GotoTag=I_Cn_Db_EMT  TagVisibility=global
  From9 : From  Commented=on  GotoTag=An_Icap
  From92 : From  Commented=on  GotoTag=I_Cn_Dt_EMT  TagVisibility=global
  From93 : From  Commented=on  GotoTag=I_Cp_Db_EMT  TagVisibility=global
  From94 : From  Commented=on  GotoTag=I_Cp_Dt_EMT  TagVisibility=global
  From95 : From  Commented=on  GotoTag=I_Ap_Db_EMT  TagVisibility=global
  From96 : From  Commented=on  GotoTag=Uref_Ap  TagVisibility=global
  From97 : From  Commented=on  GotoTag=I_Ap_Dt_EMT  TagVisibility=global
  From99 : From  Commented=on  GotoTag=IBRK
  Gain : Gain  Commented=on  Gain=0
  Gain1 : Gain  Commented=on  Gain=-1
  Gain2 : Gain  Commented=on  Gain=D_Rs/(D_R+D_Rs)
  Gain3 : Gain  Commented=on
  Gain4 : Gain  Commented=on  Gain=1/Vb_dc
  Gain5 : Gain  Gain=2*pi*50
  Gain6 : Gain  Commented=on  Gain=0.5
  Gain7 : Gain  Commented=on  Gain=1/Vb_dc
  Gain8 : Gain
  Gates1 : Subsystem
  Goto : Goto  Commented=on  GotoTag=IBrk2_EMT  TagVisibility=global
  Goto1 : Goto  Commented=on  GotoTag=IBrk1_EMT  TagVisibility=global
  Goto10 : Goto  Commented=on  GotoTag=Vdc_ss
  Goto11 : Goto  Commented=on  GotoTag=Id_ss  TagVisibility=global
  Goto114 : Goto  Commented=on  GotoTag=uns
  Goto116 : Goto  Commented=on  GotoTag=u_zero
  Goto12 : Goto  Commented=on  GotoTag=UBrk2_EMT  TagVisibility=global
  Goto13 : Goto  Commented=on  GotoTag=UBrk1_EMT  TagVisibility=global
  Goto14 : Goto  Commented=on  GotoTag=UBrk2_EMT  TagVisibility=global
  Goto15 : Goto  Commented=on  GotoTag=UBrk1_EMT  TagVisibility=global
  Goto16 : Goto  Commented=on  GotoTag=U_An_Db
  Goto17 : Goto  Commented=on  GotoTag=U_An_Dt
  Goto18 : Goto  Commented=on  GotoTag=U_Bp_Dt
  Goto19 : Goto  Commented=on  GotoTag=U_Cn_Db
  Goto2 : Goto  Commented=on  GotoTag=UBrk1_ss
  Goto22 : Goto  Commented=on  GotoTag=U_Cn_Dt
  Goto23 : Goto  Commented=on  GotoTag=U_An_ss
  Goto24 : Goto  Commented=on  GotoTag=U_Ap_ss
  Goto25 : Goto  Commented=on  GotoTag=U_Bn_ss
  Goto27 : Goto  Commented=on  GotoTag=U_Bp_ss
  Goto28 : Goto  Commented=on  GotoTag=U_Cn_ss
  Goto3 : Goto  Commented=on  GotoTag=UBrk2_ss
  Goto30 : Goto  Commented=on  GotoTag=Uref_ABC_ss
  Goto31 : Goto  Commented=on  GotoTag=U_Cp_ss
  Goto32 : Goto  Commented=on  GotoTag=U_Cp_Db
  Goto33 : Goto  Commented=on  GotoTag=U_Cp_Dt
  Goto34 : Goto  Commented=on  GotoTag=Uref_Bn_ss  TagVisibility=global
  Goto36 : Goto  Commented=on  GotoTag=U_Ap_Db
  Goto37 : Goto  Commented=on  GotoTag=U_Ap_Dt
  Goto38 : Goto  Commented=on  GotoTag=U_Bn_Db
  Goto39 : Goto  Commented=on  GotoTag=U_Bn_Dt
  Goto4 : Goto  Commented=on  GotoTag=Vprim_ss
  Goto40 : Goto  Commented=on  GotoTag=U_Bp_Db
  Goto41 : Goto  Commented=on  GotoTag=Iprim_ss
  Goto42 : Goto  Commented=on  GotoTag=Isec_ss
  Goto43 : Goto  Commented=on  GotoTag=An_Icap
  Goto44 : Goto  Commented=on  GotoTag=An_Ipos
  Goto45 : Goto  Commented=on  GotoTag=Ap_Icap
  Goto46 : Goto  Commented=on  GotoTag=Ap_Ipos
  Goto47 : Goto  Commented=on  GotoTag=Bn_Icap
  Goto48 : Goto  Commented=on  GotoTag=Bn_Ipos
  Goto49 : Goto  Commented=on  GotoTag=Bp_Icap
  Goto5 : Goto  Commented=on  GotoTag=Vsec_ss
  Goto50 : Goto  Commented=on  GotoTag=Bp_Ipos
  Goto51 : Goto  Commented=on  GotoTag=Cn_Icap
  Goto52 : Goto  Commented=on  GotoTag=Cn_Ipos
  Goto53 : Goto  Commented=on  GotoTag=Cp_Icap
  Goto54 : Goto  Commented=on  GotoTag=Cp_Ipos
  Goto56 : Goto  Commented=on  GotoTag=Ip_ss
  Goto58 : Goto  Commented=on  GotoTag=In_ss
  Goto59 : Goto  Commented=on  GotoTag=Vprim_ss
  Goto6 : Goto  Commented=on  GotoTag=Iprim_ss
  Goto60 : Goto  Commented=on  GotoTag=Vsec_ss
  Goto61 : Goto  Commented=on  GotoTag=Ip_ss
  Goto62 : Goto  Commented=on  GotoTag=In_ss
  Goto63 : Goto  Commented=on  GotoTag=Idc1p_ss
  Goto64 : Goto  Commented=on  GotoTag=Idc1n_ss
  Goto65 : Goto  Commented=on  GotoTag=Idc1p_ss
  Goto66 : Goto  Commented=on  GotoTag=Idc1n_ss
  Goto67 : Goto  Commented=on  GotoTag=Vdc_ss
  Goto68 : Goto  Commented=on  GotoTag=Id_ss
  Goto69 : Goto  Commented=on  GotoTag=Uref_An_ss  TagVisibility=global
  Goto7 : Goto  Commented=on  GotoTag=Isec_ss
  Goto70 : Goto  Commented=on  GotoTag=Uref_Cn_ss  TagVisibility=global
  Goto71 : Goto  Commented=on  GotoTag=An_Vbl_ss
  Goto72 : Goto  Commented=on  GotoTag=An_Vin_ss
  Goto73 : Goto  Commented=on  GotoTag=Uref_Bp_ss  TagVisibility=global
  Goto74 : Goto  Commented=on  GotoTag=Uref_Ap_ss  TagVisibility=global
  Goto75 : Goto  Commented=on  GotoTag=Uref_Cp_ss  TagVisibility=global
  Goto76 : Goto  Commented=on  GotoTag=Ap_Vbl_ss
  Goto77 : Goto  Commented=on  GotoTag=Ap_Vin_ss
  Goto78 : Goto  Commented=on  GotoTag=Bn_Vbl_ss
  Goto79 : Goto  Commented=on  GotoTag=Bn_Vin_ss
  Goto8 : Goto  Commented=on  GotoTag=Idc1p_ss
  Goto80 : Goto  Commented=on  GotoTag=Bp_Vbl_ss
  Goto81 : Goto  Commented=on  GotoTag=Bp_Vin_ss
  Goto82 : Goto  Commented=on  GotoTag=Cn_Vbl_ss
  Goto83 : Goto  Commented=on  GotoTag=Cn_Vin_ss
  Goto84 : Goto  Commented=on  GotoTag=Cp_Vbl_ss
  Goto85 : Goto  Commented=on  GotoTag=Cp_Vin_ss
  Goto86 : Goto  Commented=on  GotoTag=u
  Goto9 : Goto  Commented=on  GotoTag=Idc1n_ss
  Ground2 : spsGroundLib/Ground  Commented=on  LConnTagsString=a
  I->pu1 : Gain  Commented=on  Gain=0.5  SaturateOnIntegerOverflow=on  OutDataTypeStr=Inherit: Same as input  ParamDataTypeStr=Inherit: Same as input
  I->pu3 : Gain  Commented=on  Gain=0.5  SaturateOnIntegerOverflow=on  OutDataTypeStr=Inherit: Same as input  ParamDataTypeStr=Inherit: Same as input
  Ld1 : spsThreePhaseSeriesRLCLoadLib/Three-Phase Series RLC Load  LConnTagsString=A|B|C  Configuration=Y (grounded)  NominalVoltage=Vnom_prim  Vabc=[1e3 1e3 1e3]  Vabcp=[1e3 1e3 1e3]  NominalFrequency=Fnom  UnbalancedPower=off  ActivePower=P_Ld1  InductivePower=0  CapacitivePower=0  Pabc=[10e3 9e3 11e3]  QLabc=[100 90 110]  QCabc=[100 90 110]  Pabcp=[10e3 9e3 11e3]  QLabcp=[100 90 110]  QCabcp=[100 90 110]  Measurements=None  LoadType=constant Z
  Ld2 : spsThreePhaseSeriesRLCLoadLib/Three-Phase Series RLC Load  LConnTagsString=A|B|C  Configuration=Y (grounded)  NominalVoltage=Vnom_sec  Vabc=[1e3 1e3 1e3]  Vabcp=[1e3 1e3 1e3]  NominalFrequency=Fnom  UnbalancedPower=off  ActivePower=500e3  InductivePower=0  CapacitivePower=0  Pabc=[10e3 9e3 11e3]  QLabc=[100 90 110]  QCabc=[100 90 110]  Pabcp=[10e3 9e3 11e3]  QLabcp=[100 90 110]  QCabcp=[100 90 110]  Measurements=None  LoadType=constant Z
  MATLAB Function : MATLAB Function  Commented=on  TreatAsAtomicUnit=on
  MATLAB Function1 : MATLAB Function  Commented=on  TreatAsAtomicUnit=on  mask{Ad=ACDC3.Adiscrete, Bd=ACDC3.Bdiscrete, Cd=ACDC3.Cdiscrete, Dd=ACDC3.Ddiscrete, InitVec=ACDC3.x0, dt=Ts_Power, nsw=6}
      mask prompts: Ad "A"; Bd "B"; Cd "C"; Dd "D"; InitVec "Initial values:"; dt "Time step (s):"; nsw "Number of switches:"
  MATLAB Function2 : MATLAB Function  Commented=on  SystemSampleTime=Ts_Power  mask{Ts=Ts_Power, D_R=D_R, D_Rs=D_Rs, Nb_SM=Nb_PM, C=C_PM}
      mask prompts: Ts "Time step (s):"; D_R "Resistance Ron (Ohms):"; D_Rs "Snubber resistance Rs (Ohms):"; Nb_SM "Number of submodules:"; C "Submodule capacitance (F):"
      settings: MinAlgLoopOccurrences=on
  MATLAB Function3 : MATLAB Function  Commented=on  TreatAsAtomicUnit=on  mask{Ad=S.A, Bd=S.B, Cd=S.C, Dd=S.D, swOnRes=S.SwitchResistance, swOffRes=1e6*ones(20,1), swType=S.SwitchType, InitVec=ACDC.x0, dt=Ts_Power, nrSWvec=[8 12]}
      mask prompts: Ad "A"; Bd "B"; Cd "C"; Dd "D"; swOnRes "Switch on resistance:"; swOffRes "Switch off resistance:"; swType "Switch type:"; InitVec "Initial values:"; dt "Time step (s):"; nrSWvec "Number of switches:"
  MATLAB Function4 : MATLAB Function  Commented=on  TreatAsAtomicUnit=on  mask{Ad=ACDC.Adiscrete, Bd=ACDC.Bdiscrete, Cd=ACDC.Cdiscrete, Dd=ACDC.Ddiscrete, swOnRes=0.001*ones(20,1), swOffRes=1e6*ones(20,1), swType=[ones(2,1); 2*ones(6,1); 3*ones(12,1)], InitVec=ACDC.x0, dt=Ts_Power, nrSWvec=[8 12]}
      mask prompts: Ad "A"; Bd "B"; Cd "C"; Dd "D"; swOnRes "Switch on resistance:"; swOffRes "Switch off resistance:"; swType "Switch type:"; InitVec "Initial values:"; dt "Time step (s):"; nrSWvec "Number of switches:"
  MATLAB Function5 : MATLAB Function  TreatAsAtomicUnit=on  mask{Ad=S.A, Bd=S.B, Cd=S.C, Dd=S.D, swOnRes=S.SwitchResistance, swOffRes=1e6*ones(20,1), swType=S.SwitchType, InitVec=ACDC.x0, dt=Ts_Power, nrSWvec=[8 12]}
      mask prompts: Ad "A"; Bd "B"; Cd "C"; Dd "D"; swOnRes "Switch on resistance:"; swOffRes "Switch off resistance:"; swType "Switch type:"; InitVec "Initial values:"; dt "Time step (s):"; nrSWvec "Number of switches:"
  MMC : Subsystem  Commented=on
  MMC1 : Subsystem
  MMC_SS : Subsystem  Commented=on
  Model1 : Subsystem  Commented=on  AncestorBlock=spsDiodeModel/Discrete  mask(DiscreteModel){}
  Model2 : Subsystem  Commented=on  AncestorBlock=spsDiodeModel/Discrete  mask(DiscreteModel){}
  Multimeter : spsMultimeterLib/Multimeter  Commented=on  L=12  sel=[7 8 9 10 11 12]  yselected={}  Gain=[1 1 1 1 1 1]  OutputType=Complex  PlotAtSimulationStop=off  PhasorSimulation=off
  Multimeter1 : spsMultimeterLib/Multimeter  Commented=on  L=12  sel=[1 2 3 4 5 6]  yselected={}  Gain=[1 1 1 1 1 1]  OutputType=Complex  PlotAtSimulationStop=off  PhasorSimulation=off
  Multimeter2 : spsMultimeterLib/Multimeter  Commented=on  L=12  sel=[1 2 3 4 5 6]  yselected={}  Gain=[1 1 1 1 1 1]  OutputType=Complex  PlotAtSimulationStop=off  PhasorSimulation=off
  Mux{,1..7,12,14,18,22,26..27,37,47,50} (17 alike) : Mux  Commented=on  Inputs=3
  Mux{8..11,13,24,28,32..35,38..43} (17 alike) : Mux  Commented=on  Inputs=2
  Mux15 : Mux  Commented=on  Inputs=numel(ACDC.inputs)
  Mux16 : Mux  Inputs=8
  Mux17 : Mux  Inputs=3
  Mux19 : Mux  Inputs=3
  Mux{20,48..49,51..55,58..60} (11 alike) : Mux  Inputs=2
  Mux21 : Mux  Inputs=3
  Mux23 : Mux  Commented=on  Inputs=numel(ACDC3.inputs)
  Mux25 : Mux  Commented=on
  Mux29 : Mux  Commented=on  Inputs=5
  Mux30 : Mux  Commented=on  Inputs=5
  Mux31 : Mux  Commented=on
  Mux36 : Mux  Commented=on  Inputs=12
  Mux44 : Mux  Commented=on
  Mux45 : Mux  Commented=on  Inputs=[1 1 1 1 1 1 1 1 1 1 1 1 1 1 1 1 1]
  Mux46 : Mux  Commented=on  Inputs=13
  Mux56 : Mux  Inputs=12
  Mux57 : Mux  Inputs=6
  Mux_u : Mux  Commented=on  Inputs=[20 17]
  P (MW) : Display  Commented=on
      settings: Format=bank  Decimation=5000
  Q (Mvar) : Display  Commented=on
      settings: Format=bank  Decimation=5000
  RL Src : spsThreePhaseSeriesRLCBranchLib/Three-Phase Series RLC Branch  LConnTagsString=A|B|C  RConnTagsString=A|B|C  BranchType=RL  Resistance=0.8929  Inductance=16.58e-3  Capacitance=1e-6  Measurements=None
  R_startup : spsThreePhaseSeriesRLCBranchLib/Three-Phase Series RLC Branch  LConnTagsString=A|B|C  RConnTagsString=A|B|C  BranchType=R  Resistance=R_startup  Inductance=Vnom_prim^2 / Pcc / (2*pi*Fnom)  Capacitance=1e-6  Measurements=None
  Rate Transition{,1..5} (6 alike) : RateTransition  Commented=on
  Scope : Scope  Commented=on  NumInputPorts=2
  Scope1 : Scope  Commented=on  NumInputPorts=2
  Scope13 : Scope  Commented=on  NumInputPorts=3
  Scope2 : Scope  Commented=on  NumInputPorts=5
  Scope3 : Scope  Commented=on  NumInputPorts=4
  Scope4 : Scope  NumInputPorts=2
  Scope5 : Scope  Commented=on  NumInputPorts=4
  Scope6 : Scope  NumInputPorts=2
  Scope7 : Scope  Commented=on
  Scope8 : Scope  NumInputPorts=2
  Scopes & Measurements : Subsystem
  Selector1 : Selector  InputPortWidth=52  IndexOptions=Index vector (dialog)  Indices=[50:52]  OutputSizes=1
  Selector10 : Selector  InputPortWidth=52  IndexOptions=Index vector (dialog)  Indices=[28:30]  OutputSizes=1
  Selector{11..16} (6 alike) : Selector  InputPortWidth=3  IndexOptions=Index vector (dialog)  Indices=1  OutputSizes=1
  Selector2 : Selector  InputPortWidth=52  IndexOptions=Index vector (dialog)  Indices=[50:52]  OutputSizes=1
  Selector3 : Selector  InputPortWidth=20  IndexOptions=Index vector (dialog)  Indices=[1:8]  OutputSizes=1
  Selector4 : Selector  InputPortWidth=52  IndexOptions=Index vector (dialog)  Indices=[9:20]  OutputSizes=1
  Selector5 : Selector  InputPortWidth=52  IndexOptions=Index vector (dialog)  Indices=[9:20]  OutputSizes=1
  Selector6 : Selector  InputPortWidth=52  IndexOptions=Index vector (dialog)  Indices=[35:46]  OutputSizes=1
  Selector7 : Selector  InputPortWidth=52  IndexOptions=Index vector (dialog)  Indices=[35:46]  OutputSizes=1
  Selector8 : Selector  InputPortWidth=17  IndexOptions=Index vector (dialog)  Indices=[3:14]  OutputSizes=1
  Selector9 : Selector  InputPortWidth=52  IndexOptions=Index vector (dialog)  Indices=[28:30]  OutputSizes=1
  Sequencer : Subsystem
      mask Display: disp('Sequencer')
  Sources : Subsystem
  State-Space1 : S-Function  FunctionName=sfun_spssw_discc  Parameters=S.Ts,S.A, S.B, S.C, S.D, S.x0, S.EnableUseOfTLC,S.SwitchResistance ,S.SwitchType, S.SwitchGateInitialValue, S.OutputsToResetToZero, S.TBEON,S.SaveMatrices,S.BufferSize  SFunctionDeploymentMode=off  EnableBusSupport=off
  Status : From  Commented=on  GotoTag=T43_3835_2986319703090  TagVisibility=global
      settings: CloseFcn=tagdialog Close
  Status_Bottom : From  Commented=on  GotoTag=T42_3768_2839018950081  TagVisibility=global
      settings: CloseFcn=tagdialog Close
  Status_Top : From  Commented=on  GotoTag=T43_3835_2986319703090  TagVisibility=global
      settings: CloseFcn=tagdialog Close
  Subtract : Sum  Commented=on  Inputs=+-
  Sum : Sum  Commented=on  Inputs=|++
  Sum2 : Sum  Commented=on  Inputs=|+-
  Sum23 : Sum  Commented=on  Inputs=|++
  Sum25 : Sum  Commented=on  Inputs=|++
  SwitchCurrents : Constant  Commented=on  Value=zeros(20,1)
  To Workspace : ToWorkspace  VariableName=ysim  SampleTime=Ts_Power
      settings: Save2DSignal=2-D array (concatenate along first dimension)
  To Workspace1 : ToWorkspace  Commented=on  VariableName=bvecsim  SampleTime=Ts_Power
      settings: Save2DSignal=2-D array (concatenate along first dimension)
  To Workspace2 : ToWorkspace  VariableName=usim  SampleTime=Ts_Power
      settings: Save2DSignal=2-D array (concatenate along first dimension)
  To Workspace3 : ToWorkspace  VariableName=bsim  SampleTime=Ts_Power
      settings: Save2DSignal=2-D array (concatenate along first dimension)
  To Workspace4 : ToWorkspace  VariableName=ssim  SampleTime=Ts_Power
      settings: Save2DSignal=2-D array (concatenate along first dimension)
  To Workspace5 : ToWorkspace  Commented=on  VariableName=idsim1  SampleTime=Ts_Power
      settings: Save2DSignal=2-D array (concatenate along first dimension)
  To Workspace6 : ToWorkspace  Commented=on  VariableName=idsim  SampleTime=Ts_Power
      settings: Save2DSignal=2-D array (concatenate along first dimension)
  Tr1 : spsThreePhaseTransformerTwoWindingsLib/Three-Phase Transformer (Two Windings)  Winding1Connection=Yg  Winding2Connection=Yg  CoreType=Three single-phase transformers  SetSaturation=off  Hysteresis=off  DataFile='hysteresis'  SetInitialFlux=off  Measurements=None  UNITS=pu  NominalPower=[ Pnom , Fnom ]  Winding1="[ Vnom_prim , Rxfo/2,  Lxfo/2 ]"  Winding2="[ Vnom_sec , Rxfo/2,  Lxfo/2 ]"  Rm=1000  Lm=1000  L0=0.5  Saturation=[ 0,0 ; 0.0024,1.2 ; 1.0,1.52 ]  InitialFluxes=[ 0.8 , -0.8 , 0.7 ]  BreakLoop=off  DiscreteSolver=Trapezoidal iterative  DataType=off  TransfoNumber=1
  USW_Bottom : From  Commented=on  GotoTag=T43_3867_2942891286788  TagVisibility=global
  USW_Bottom1 : From  Commented=on  GotoTag=T43_3867_2942891286788  TagVisibility=global
  USW_Top2 : From  Commented=on  GotoTag=T44_3934_3096165412659  TagVisibility=global
  USW_Top3 : From  Commented=on  GotoTag=T44_3934_3096165412659  TagVisibility=global
  Uref2m1 : Subsystem  Commented=on
  Uref2m2 : Subsystem  Commented=on
  Uref2m3 : Subsystem
  V1 (kV rms LL) : Display  Commented=on
      settings: Format=bank  Decimation=5000
  VS Conv2b : spsControlledVoltageSourceLib/Controlled Voltage Source  Commented=on  Initialize=on  Source_Type=AC  Amplitude=0  Phase=0  Frequency=0  Measurements=None
  VS Conv2t : spsControlledVoltageSourceLib/Controlled Voltage Source  Commented=on  Initialize=on  Source_Type=AC  Amplitude=0  Phase=0  Frequency=0  Measurements=None
  Vdc (kV) : Display  Commented=on
      settings: Format=bank  Decimation=5000
  Voltage source : Subsystem
  Voltage source1 : Subsystem  Commented=on
  param : Subsystem  Commented=on
      settings: OpenFcn=open('HVDCMMCInterconnectionParam')
      mask Display: disp('Double-click to open\nparameters file')
  powergui : spspowerguiLib/powergui  Priority=1  SimulationMode=Discrete  SampleTime=Ts_Power  frequency=60  Iterations=50  frequencyindice=0  Pbase=100e6  ErrMax=1e-4  UnitsV=kV  UnitsW=MW  buscounter=0  FunctionMessages=off  echomessages=off  EnableUseOfTLC=off  CurrentSourceSwitches=off  DisableSnubberDevices=off  DisableRonSwitches=off  DisableVfSwitches=off  DisplayEquations=off  AutomaticDiscreteSolvers=off  SolverType=Tustin/Backward Euler (TBE)  Interpol=off  ExternalGateDelay=off  methode=off  Ts=10  x0status=blocks  SPID=off  SwTol=0  HookPort=off  NonlinearTolerance=1e-4  nMaxIteration=100  ContinueOnMaxIteration=off  RestoreLinks=warning  ResistiveCurrentMeasurement=off  Frange=[0:2:500]  Ylog=off  Xlog=on  ShowGrid=off  save=off  variable=ZData  structure=VIprim  ZoomFFT=on  StartTime=0.15  cycles=2  DisplayStyle=1  fundamental=50  FreqAxis=on  MaxFrequency=1000  frequencyindicesteady=1  RmsSteady=1  display=off
  prim : spsThreePhaseVIMeasurementLib/Three-Phase V-I Measurement  VoltageMeasurement=phase-to-ground  SetLabelV=on  LabelV=Vprim  Vpu=off  VpuLL=off  CurrentMeasurement=yes  SetLabelI=on  LabelI=Iprim  Ipu=off  Pbase=100e6  Vbase=500e3  OutputType=Complex  PhasorSimulation=off  PSBequivalent=0
  sec : spsThreePhaseVIMeasurementLib/Three-Phase V-I Measurement  VoltageMeasurement=phase-to-ground  SetLabelV=on  LabelV=Vsec  Vpu=off  VpuLL=off  CurrentMeasurement=yes  SetLabelI=on  LabelI=Isec  Ipu=off  Pbase=100e6  Vbase=500e3  OutputType=Complex  PhasorSimulation=off  PSBequivalent=0
  tag scope: Uref_ABC=global, Uref_An_d=global, Uref_Ap_d=global, Uref_Bn_d=global, Uref_Bp_d=global, Uref_Cn_d=global, Uref_Cp_d=global, Vsrc_ABC=global, meas1=global, wt0=global
  wires:
  From2/1 -> P (MW)/1
  From4/1 -> Vdc (kV)/1
  From5/1 -> V1 (kV rms LL)/1
  From11/1 -> Q (Mvar)/1
  From/1 -> Uref2m1/1(In1)
  [PQreg_On] -> Control/1(PQreg_ON)
  [Vdc_ref] -> Control/2(Vdc_ref)
  [Qref] -> Control/3(Qref)
  [Vsec] -> Control/4(Vsec)
  [Isec] -> Control/5(Isec)
  Control/1(Uref) -> [Uref_ABC]
  Control/2(Meas) -> [meas1]
  Control/3(m1_dq) -> ?
  Control/4(wt) -> ?
  [Vsrc_ABC] -> Voltage source/1(In1)
  [wt0] -> DQn->ABC/2(tho)  "theta"
  [VSRC_C] -> DQn->ABC/1(Xdcpnz_c)  "[N+1,18 (6+6+6)]"
  [Vsec] -> Scope8/2
  DQn->ABC/1(Xabc) -> Scope8/1, [Vsrc_ABC]  "Mac_EMT"
  Constant3/1 -> [VSRC_C]
  Gain5/1 -> [wt0]
  Clock/1 -> Gain5/1
  From6/1 -> Voltage source1/1(In1)
  From1/1 -> 3ph SM1/1(Uref_An)
  From7/1 -> 3ph SM1/2(An_Ipos)
  From9/1 -> 3ph SM1/3(An_Icap)
  From27/1 -> Scope2/2  "U_Ap_Dt"
  From28/1 -> Scope2/3  "U_Ap_Dt"
  From102/1 -> Gain4/1  "Ap_Vin"
  From103/1 -> Gain7/1  "Ap_Vbl"
  Status/1 -> Mux9/2  "Status"
  Gain4/1 -> Scope2/4  "Ap_Vin"
  Gain7/1 -> Scope2/5  "Ap_Vbl"
  Mux9/1 -> Scope2/1
  MATLAB Function/2(status) -> Mux9/1
  From44/1 -> MATLAB Function/1(Id)  "U_Ap_Dt"
  From39/1 -> MATLAB Function/2(Vd)  "U_Ap_Dt"
  [Converter2_On] -> Conv 2/1(On)
  ? -> Model2/1(Uswitch)  "USW_Bottom_fcn"
  ? -> Model2/2(status)  "Status_Bottom_Fcn"
  ? -> Model1/1(Uswitch)  "USW_Top"
  ? -> Model1/2(status)  "Status_Top"
  From85/1 -> 3ph SM2/3(Ap_Icap)
  From34/1 -> 3ph SM2/1(Uref_Ap)
  From36/1 -> 3ph SM2/2(Ap_Ipos)
  From91/1 -> Delay10/1  "Ap_Icap"
  From69/1 -> Delay3/1  "U_Ap_SM"
  From90/1 -> Delay11/1  "Ap_Ipos"
  Delay11/1 -> MATLAB Function2/4(Ic)
  Delay10/1 -> MATLAB Function2/3(Ip)
  Delay3/1 -> MATLAB Function2/1(Usm)
  MATLAB Function2/1(UDt) -> Mux24/2  "USW_Top_fcn"
  USW_Top2/1 -> Mux24/1  "USW_Top"
  Mux24/1 -> Scope3/1
  Mux28/1 -> Scope3/2
  USW_Bottom/1 -> Mux28/1  "USW_Bottom"
  MATLAB Function2/3(UDb) -> Mux28/2  "USW_Bottom_fcn"
  Mux29/1 -> Scope3/3
  Status_Top/1 -> Mux29/1  "Status_Top"
  MATLAB Function2/2(Stt) -> Mux29/2  "Status_Top"
  Mux30/1 -> Scope3/4, Scope7/1
  Status_Bottom/1 -> Mux30/1  "Status_Bottom"
  MATLAB Function2/4(Stb) -> Mux30/2  "Status_Bottom_Fcn"
  Mux35/1 -> Scope5/4
  Mux33/1 -> Scope5/2
  Mux34/1 -> Scope5/3
  Mux32/1 -> Scope5/1
  From118/1 -> Mux35/2
  MATLAB Function2/6(IDb) -> Mux33/2  "Db_fcn"
  MATLAB Function2/5(IDt) -> Mux32/2  "Dt_fcn"
  From48/1 -> Mux32/1  "I_Ap_Dt"
  From107/1 -> Mux33/1  "I_Ap_Db"
  USW_Top3/1 -> Mux34/1  "USW_Top"
  Gain1/1 -> Mux34/2
  USW_Bottom1/1 -> Gain1/1  "USW_Bottom"
  From113/1 -> Mux35/1  "I_Ap_Dt"
  From119/1 -> Delay8/1(In1)  "Ap_Ipos"
  Delay9/1(Out1) -> Mux29/3, Subtract/1  "Ipos"
  From120/1 -> Delay9/1(In1)  "Ap_Icap"
  Delay8/1(Out1) -> Gain2/1  "Icap"
  Gain2/1 -> Mux29/4, Subtract/2
  Subtract/1 -> Mux29/5  "Ib"
  From96/1 -> MATLAB Function2/2(Uref)
  MATLAB Function1/1(y) -> Demux6/1, Demux7/1
  Mux23/1 -> MATLAB Function1/1(u), DSS1/1(U)
  Multimeter/1 -> Demux/1
  Demux/2 -> Goto/1
  Demux/1 -> Goto1/1
  Demux1/1 -> Mux23/1
  Demux1/2 -> Mux23/2
  Demux1/3 -> Mux23/3
  From8/1 -> Demux1/1
  Demux2/2 -> Mux23/5
  Demux2/3 -> Mux23/6
  Demux2/1 -> Mux23/4
  From12/1 -> Mux23/8
  From13/1 -> Mux23/7
  From14/1 -> Mux23/10
  From15/1 -> Mux23/9
  From16/1 -> Mux23/12
  From17/1 -> Mux23/11
  From114/1 -> Mux23/14
  From115/1 -> Mux23/13
  From18/1 -> Demux3/1
  Demux3/1 -> Mux23/15
  Demux3/2 -> Mux23/16
  Demux3/3 -> Mux23/17
  Demux6/3 -> Mux/3
  Demux6/2 -> Mux/2
  Demux6/1 -> Mux/1
  Mux/1 -> Mux12/2, Goto2/1
  Demux6/6 -> Mux1/3
  Demux6/4 -> Mux1/1
  Mux1/1 -> Mux14/2, Goto3/1
  Demux6/5 -> Mux1/2
  Mux4/1 -> Goto6/1
  Mux5/1 -> Goto7/1
  Mux39/1 -> Rate Transition2/1
  From204/1 -> Mux39/1  "Vsec_EMT"
  Rate Transition5/1 -> COMPARE1/6
  Rate Transition4/1 -> COMPARE1/5
  Rate Transition3/1 -> COMPARE1/4
  Rate Transition2/1 -> COMPARE1/3
  Rate Transition/1 -> COMPARE1/1
  From199/1 -> Mux39/2  "Vsec_ss"
  Gain6/1 -> Mux38/2  "Idc_ss"
  From207/1 -> Mux41/2  "Vdc_ss"
  From209/1 -> Mux43/1
  From198/1 -> Mux42/2  "Idiff_ss"
  Add1/1 -> Gain6/1
  Rate Transition1/1 -> COMPARE1/2
  From65/1 -> Mux40/1  "Isec_EMT"
  Mux42/1 -> Rate Transition4/1
  From200/1 -> Mux42/1  "Idiff_EMT"
  From201/1 -> Add1/1
  From210/1 -> Mux43/2
  Mux38/1 -> Rate Transition/1
  From208/1 -> Mux41/1  "Vdc_EMT"
  Mux40/1 -> Rate Transition3/1
  From202/1 -> Add1/2
  From203/1 -> Mux38/1  "Idc_EMT"
  Mux41/1 -> Rate Transition1/1
  From206/1 -> Mux40/2  "Isec_ss"
  Mux43/1 -> Rate Transition5/1
  Mux6/1 -> Goto56/1
  Mux7/1 -> Goto58/1
  Demux6/13 -> Goto31/1
  Mux2/1 -> Goto4/1
  Demux6/12 -> Goto28/1
  Demux6/11 -> Goto27/1
  Demux6/9 -> Goto24/1
  Demux6/14 -> Mux2/1
  Demux6/15 -> Mux2/2
  Demux6/8 -> Goto23/1
  Demux6/10 -> Goto25/1
  Demux6/16 -> Mux2/3
  Mux3/1 -> Goto5/1
  Demux6/7 -> Goto10/1
  I->pu1/1 -> Goto11/1
  From20/1 -> Sum2/1
  Sum2/1 -> I->pu1/1  "Idiff"
  From22/1 -> Sum2/2
  Demux6/17 -> Mux3/1
  Demux6/18 -> Mux3/2
  Demux6/19 -> Mux3/3
  Demux6/20 -> Goto9/1
  Demux6/21 -> Goto8/1
  Demux6/33 -> Mux5/3
  Demux6/32 -> Mux5/2
  Demux6/31 -> Mux5/1
  Demux6/30 -> Mux4/3
  Demux6/29 -> Mux4/2
  Demux6/28 -> Mux4/1
  Demux6/22 -> Mux7/1
  Demux6/24 -> Mux7/2
  Demux6/26 -> Mux7/3
  Demux6/23 -> Mux6/1
  Demux6/25 -> Mux6/2
  Demux6/27 -> Mux6/3
  From10/1 -> Demux2/1
  From26/1 -> Mux13/1  "UBrk1_EMT"
  From33/1 -> Mux13/2  "UBrk2_EMT"
  Multimeter1/1 -> Demux4/1
  Demux4/1 -> Goto13/1, BRK_CTRL/1(UBrk1_EMT)  "UBrk1_EMT"
  From25/1 -> BRK_CTRL/2(Brk_ON)
  From29/1 -> BRK_CTRL1/2(Brk_ON)
  Demux4/2 -> Goto12/1, BRK_CTRL1/1(UBrk1_EMT)  "UBrk2_EMT"
  Mux8/1 -> Scope/1
  Mux10/1 -> Scope/2
  From31/1 -> Mux8/1
  From30/1 -> Mux10/1
  BRK_CTRL/1(IBrk1_ss) -> Mux8/2  "IBrk1_ss"
  BRK_CTRL1/1(IBrk1_ss) -> Mux10/2  "IBrk2_ss"
  [Brk1_On] -> Brk1/1
  [Brk2_On] -> Brk2/1
  From24/1 -> Cast To Double/1
  From19/1 -> Cast To Double1/1
  Mux11/1 -> To Workspace1/1, MATLAB Function1/2(bvec)
  Cast To Double/1 -> Mux11/1
  Cast To Double1/1 -> Mux11/2
  Demux5/2 -> Goto14/1
  Demux5/1 -> Goto15/1
  Multimeter2/1 -> Demux5/1
  From35/1 -> Mux12/1
  From40/1 -> Mux14/1
  Mux12/1 -> Scope1/1
  Mux14/1 -> Scope1/2
  Demux7/1 -> Demux8/1
  Demux8/1 -> Mux12/3
  Demux8/2 -> Mux14/3
  Demux9/9 -> Goto16/1
  Demux9/16 -> Goto18/1
  Demux9/11 -> Goto36/1
  Demux9/10 -> Goto17/1
  Demux9/13 -> Goto38/1
  Demux9/19 -> Goto32/1
  Demux9/18 -> Goto22/1
  Demux9/17 -> Goto19/1
  Demux9/20 -> Goto33/1
  Demux9/14 -> Goto39/1
  Demux9/15 -> Goto40/1
  Demux9/12 -> Goto37/1
  Demux9/48 -> Mux22/2
  Demux9/51 -> Mux18/2
  Demux9/47 -> Mux22/1
  Demux9/50 -> Mux18/1
  Mux22/1 -> Goto41/1
  Demux9/49 -> Mux22/3
  Demux9/52 -> Mux18/3
  Mux18/1 -> Goto42/1
  Demux9/41 -> Goto49/1
  Demux9/39 -> Goto47/1
  Demux9/44 -> Goto52/1
  Demux9/43 -> Goto51/1
  Demux9/35 -> Goto43/1
  Demux9/45 -> Goto53/1
  Demux9/42 -> Goto50/1
  Demux9/46 -> Goto54/1
  Demux9/36 -> Goto44/1
  Demux9/37 -> Goto45/1
  Demux9/40 -> Goto48/1
  Demux9/38 -> Goto46/1
  Demux10/3 -> Mux16/5
  Demux10/1 -> Mux16/3
  [IBrk1_EMT] -> Demux10/1
  Demux11/1 -> Mux16/6
  Demux11/3 -> Mux16/8
  Demux10/2 -> Mux16/4
  [IBrk2_EMT] -> Demux11/1
  [I_Conv2SWp] -> Mux16/2
  Demux11/2 -> Mux16/7
  [I_Conv2SWn] -> Mux16/1
  Mux16/1 -> [IBRK]
  MATLAB Function3/1(y) -> Demux9/1
  From63/1 -> Gain3/1
  Gain3/1 -> MATLAB Function3/2(brkVec)
  Mux21/1 -> To Workspace3/1, [BrkVec]
  From84/1 -> Mux46/6
  From95/1 -> Mux46/4
  From94/1 -> Mux46/13
  From86/1 -> Mux46/7
  From87/1 -> Mux46/8
  From88/1 -> Mux46/9
  From89/1 -> Mux46/10
  From83/1 -> Mux46/3
  From93/1 -> Mux46/12
  Mux46/1 -> To Workspace6/1
  From82/1 -> Mux46/2
  From97/1 -> Mux46/5
  From92/1 -> Mux46/11
  From99/1 -> Mux46/1
  Mux20/1 -> Mux21/1
  Cast To Double4/1 -> Mux20/2, Mux20/1
  [Converter2_On] -> Cast To Double4/1
  Cast To Double3/1 -> Mux19/3, Mux19/2, Mux19/1
  [Brk2_On] -> Cast To Double3/1
  Mux17/1 -> Mux21/2
  Mux19/1 -> Mux21/3
  [Brk1_On] -> Cast To Double2/1
  Cast To Double2/1 -> Mux17/3, Mux17/1, Mux17/2
  From77/1 -> Mux36/10
  From72/1 -> Mux36/7
  Mux36/1 -> To Workspace5/1
  From70/1 -> Mux36/5
  From80/1 -> Mux36/3
  From71/1 -> Mux36/6
  From67/1 -> Mux36/1
  From73/1 -> Mux36/8
  From79/1 -> Mux36/12
  From74/1 -> Mux36/9
  From81/1 -> Mux36/4
  From78/1 -> Mux36/11
  From68/1 -> Mux36/2
  ? -> Mux37/1
  Mux27/1 -> Goto60/1
  Mux37/1 -> Goto61/1
  Demux9/29 -> Mux27/2
  ? -> Goto64/1
  ? -> Mux47/2
  ? -> Mux37/2
  Demux9/28 -> Mux27/1
  ? -> Goto63/1
  ? -> Mux37/3
  ? -> Mux47/3
  ? -> Mux47/1
  Demux9/26 -> Mux26/2
  Mux47/1 -> Goto62/1
  Demux9/30 -> Mux27/3
  Demux9/27 -> Mux26/3
  Mux26/1 -> Goto59/1
  Demux9/25 -> Mux26/1
  Demux9/33 -> Goto66/1
  Demux9/34 -> Goto65/1
  Demux9/21 -> Goto67/1
  From122/1 -> Sum25/2
  From121/1 -> Sum23/2
  From112/1 -> Sum/2
  Mux50/1 -> I->pu3/1
  I->pu3/1 -> Goto68/1
  From109/1 -> Sum23/1
  Sum23/1 -> Mux50/2
  From110/1 -> Sum/1
  Sum25/1 -> Mux50/3
  From111/1 -> Sum25/1
  Sum/1 -> Mux50/1  "Idiff"
  Control1/2(Meas) -> ?
  From106/1 -> Control1/5(Isec)
  From53/1 -> Control1/4(Vsec)
  Control1/3(m1_dq) -> ?
  From105/1 -> Control1/3(Qref)
  Control1/4(wt) -> ?
  From100/1 -> Control1/1(PQreg_ON)
  From104/1 -> Control1/2(Vdc_ref)
  Control1/1(Uref) -> Goto30/1
  Uref2m2/2(Uref_Bp) -> Goto73/1
  From76/1 -> Uref2m2/2(Block)
  Uref2m2/1(Uref_Ap) -> Goto74/1
  Uref2m2/6(Uref_Cn) -> Goto70/1
  Uref2m2/3(Uref_Cp) -> Goto75/1
  Uref2m2/4(Uref_An) -> Goto69/1
  From75/1 -> Uref2m2/1(Uref_ABC)
  Uref2m2/5(Uref_Bn) -> Goto34/1
  From134/1 -> 3ph SM8/2(An_Ipos)
  From124/1 -> 3ph SM5/1(Uref_An)
  From125/1 -> 3ph SM5/2(An_Ipos)
  From126/1 -> 3ph SM5/3(An_Icap)
  From51/1 -> 3ph SM3/3(An_Icap)
  From49/1 -> 3ph SM3/2(An_Ipos)
  From47/1 -> 3ph SM3/1(Uref_An)
  From108/1 -> 3ph SM4/1(Uref_An)
  From123/1 -> 3ph SM4/3(An_Icap)
  From117/1 -> 3ph SM4/2(An_Ipos)
  From131/1 -> 3ph SM7/2(An_Ipos)
  From133/1 -> 3ph SM8/1(Uref_An)
  From135/1 -> 3ph SM8/3(An_Icap)
  From129/1 -> 3ph SM6/3(An_Icap)
  From130/1 -> 3ph SM7/1(Uref_An)
  From127/1 -> 3ph SM6/1(Uref_An)
  From132/1 -> 3ph SM7/3(An_Icap)
  From128/1 -> 3ph SM6/2(An_Ipos)
  From54/1 -> Mux25/4
  From55/1 -> Mux25/3
  Mux25/1 -> Scope13/1
  3ph SM3/2(An_Vin) -> Goto72/1
  3ph SM3/1(An_Vbl) -> Goto71/1
  3ph SM4/1(An_Vbl) -> Goto76/1
  3ph SM4/2(An_Vin) -> Goto77/1
  From64/1 -> Mux25/1
  From66/1 -> Mux25/2
  3ph SM6/1(An_Vbl) -> Goto80/1
  3ph SM5/1(An_Vbl) -> Goto78/1
  3ph SM5/2(An_Vin) -> Goto79/1
  3ph SM6/2(An_Vin) -> Goto81/1
  3ph SM8/1(An_Vbl) -> Goto84/1
  3ph SM7/1(An_Vbl) -> Goto82/1
  3ph SM7/2(An_Vin) -> Goto83/1
  3ph SM8/2(An_Vin) -> Goto85/1
  From138/1 -> Mux31/1
  From136/1 -> Mux31/4
  From139/1 -> Mux31/2
  Mux31/1 -> Scope13/2
  From137/1 -> Mux31/3
  From142/1 -> Mux44/1
  Mux44/1 -> Scope13/3
  From143/1 -> Mux44/2
  From141/1 -> Mux44/3
  From140/1 -> Mux44/4
  Mux_u/1 -> Goto86/1, MATLAB Function3/1(u)
  SwitchCurrents/1 -> Goto116/1, Mux_u/1
  Mux45/1 -> Goto114/1, Mux_u/2
  From154/1 -> Mux45/11
  From155/1 -> Mux45/14
  From153/1 -> Mux45/12
  From149/1 -> Mux45/10
  From156/1 -> Mux45/13
  From150/1 -> Mux45/9
  From151/1 -> Mux45/6
  From147/1 -> Mux45/8
  From146/1 -> Mux45/3
  From152/1 -> Mux45/5
  From148/1 -> Mux45/7
  Demux14/1 -> Mux45/15
  Constant1/1 -> Mux45/1, Mux45/2
  Demux14/2 -> Mux45/16
  From145/1 -> Mux45/4
  Demux14/3 -> Mux45/17
  From144/1 -> Demux14/1
  From179/1 -> Mux15/31
  From180/1 -> Mux15/34
  From178/1 -> Mux15/32
  From168/1 -> Mux15/30
  From181/1 -> Mux15/33
  From169/1 -> Mux15/29
  From174/1 -> Mux15/26
  From166/1 -> Mux15/28
  From165/1 -> Mux15/23
  From175/1 -> Mux15/25
  From167/1 -> Mux15/27
  From164/1 -> Mux15/24
  Demux13/8 -> Mux15/8
  Demux13/6 -> Mux15/6
  Demux12/1 -> Mux15/35
  Gain/1 -> Demux13/1
  Demux13/1 -> Mux15/1
  Demux13/3 -> Mux15/3
  Demux13/5 -> Mux15/5
  Constant2/1 -> Mux15/22, Mux15/21
  Demux13/4 -> Mux15/4
  Demux12/2 -> Mux15/36
  Mux15/1 -> ?
  From56/1 -> Gain/1
  Demux13/2 -> Mux15/2
  Demux13/7 -> Mux15/7
  Demux12/3 -> Mux15/37
  From116/1 -> Demux12/1
  State-Space1/2 -> Demux15/1, To Workspace4/1
  State-Space1/1 -> Selector6/1, Selector4/1, Selector9/1, Selector1/1, To Workspace/1
  [u_disc] -> To Workspace2/1, MATLAB Function5/1(u), State-Space1/1
  Mux55/1 -> Selector3/1, State-Space1/2
  MATLAB Function5/1(y) -> Selector10/1, Selector2/1, Selector5/1, Selector7/1
  MATLAB Function5/2(status) -> Demux16/1
  Mux54/1 -> COMPARE2/6
  Mux53/1 -> COMPARE2/5
  Mux51/1 -> COMPARE2/4
  Mux48/1 -> COMPARE2/1
  Mux49/1 -> COMPARE2/3
  Mux52/1 -> COMPARE2/2
  Demux15/1 -> Mux48/1
  Demux16/1 -> Mux48/2
  Demux16/9 -> Mux49/2
  Demux15/9 -> Mux49/1
  Demux16/10 -> Mux51/2
  Demux15/10 -> Mux51/1
  Demux16/15 -> Mux53/2
  Demux15/15 -> Mux53/1
  Demux15/20 -> Mux54/1
  Demux16/20 -> Mux54/2
  Demux15/5 -> Mux52/1
  Demux16/5 -> Mux52/2
  [BrkVec] -> Gain8/1
  Selector3/1 -> MATLAB Function5/2(brkVec)
  [BrkVec] -> Mux55/1
  Constant/1 -> Mux55/2
  Selector4/1 -> [Udiode]
  Demux17/6 -> [Bn_Ipos]
  Demux17/10 -> [Cn_Ipos]
  Demux17/9 -> [Cn_Icap]
  Demux17/1 -> [An_Icap]
  Demux17/12 -> [Cp_Ipos]
  Demux17/11 -> [Cp_Icap]
  Demux17/3 -> [Ap_Icap]
  Demux17/2 -> [An_Ipos]
  Demux17/4 -> [Ap_Ipos]
  Demux17/5 -> [Bn_Icap]
  Demux17/7 -> [Bp_Icap]
  Demux17/8 -> [Bp_Ipos]
  Selector6/1 -> [Idiode]
  Selector7/1 -> [Idiode_ss]
  [Idiode_ss] -> Scope4/2
  [Uref_Ap_d] -> 3ph SM10/1(Uref_An)
  3ph SM11/2(An_Vin) -> [Bn_Vin_ss]
  [An_Icap] -> 3ph SM9/3(An_Icap)
  [Ap_Icap] -> 3ph SM10/3(An_Icap)
  [Bp_Ipos] -> 3ph SM12/2(An_Ipos)
  [Cn_Ipos] -> 3ph SM13/2(An_Ipos)
  [Uref_Cn_d] -> 3ph SM13/1(Uref_An)
  [Uref_Bn_d] -> 3ph SM11/1(Uref_An)
  [Cp_Icap] -> 3ph SM14/3(An_Icap)
  [Cp_Ipos] -> 3ph SM14/2(An_Ipos)
  3ph SM9/2(An_Vin) -> [An_Vin_ss]
  3ph SM14/2(An_Vin) -> [Cp_Vin_ss]
  3ph SM10/2(An_Vin) -> [Ap_Vin_ss]
  3ph SM10/1(An_Vbl) -> [Ap_Vbl_ss]
  [Uref_Cp_d] -> 3ph SM14/1(Uref_An)
  3ph SM12/2(An_Vin) -> [Bp_Vin_ss]
  3ph SM13/2(An_Vin) -> [Cn_Vin_ss]
  3ph SM11/1(An_Vbl) -> [Bn_Vbl_ss]
  [Ap_Ipos] -> 3ph SM10/2(An_Ipos)
  3ph SM12/1(An_Vbl) -> [Bp_Vbl_ss]
  3ph SM14/1(An_Vbl) -> [Cp_Vbl_ss]
  [Uref_An_d] -> 3ph SM9/1(Uref_An)
  [Bp_Icap] -> 3ph SM12/3(An_Icap)
  [An_Ipos] -> 3ph SM9/2(An_Ipos)
  [Bn_Icap] -> 3ph SM11/3(An_Icap)
  3ph SM9/1(An_Vbl) -> [An_Vbl_ss]
  3ph SM13/1(An_Vbl) -> [Cn_Vbl_ss]
  [Bn_Ipos] -> 3ph SM11/2(An_Ipos)
  [Uref_Bp_d] -> 3ph SM12/1(Uref_An)
  [Cn_Icap] -> 3ph SM13/3(An_Icap)
  [An_Vbl_ss] -> Mux56/1
  [An_Vin_ss] -> Mux56/2
  [Ap_Vbl_ss] -> Mux56/3
  [Ap_Vin_ss] -> Mux56/4
  [Bn_Vbl_ss] -> Mux56/5
  [Bn_Vin_ss] -> Mux56/6
  [Bp_Vbl_ss] -> Mux56/7
  [Bp_Vin_ss] -> Mux56/8
  [Cn_Vbl_ss] -> Mux56/9
  [Cn_Vin_ss] -> Mux56/10
  [Cp_Vbl_ss] -> Mux56/11
  [Cp_Vin_ss] -> Mux56/12
  [uns] -> Selector8/1
  [Vsrc_ABC] -> Demux18/1
  Mux56/1 -> Mux57/3
  Demux18/1 -> Mux57/4
  Demux18/2 -> Mux57/5
  Demux18/3 -> Mux57/6
  Constant4/1 -> Mux57/2, Mux57/1
  Mux57/1 -> [uns_disc]
  [u_zero] -> Mux58/1
  [uns_disc] -> Mux58/2
  Mux58/1 -> [u_disc]
  Selector2/1 -> Selector16/1
  [Isec] -> Selector14/1
  Uref2m3/4(Uref_An) -> [Uref_An_d]
  Uref2m3/6(Uref_Cn) -> [Uref_Cn_d]
  Selector1/1 -> Control2/5(Isec), Selector15/1
  [Vdc_ref] -> Control2/2(Vdc_ref)
  Uref2m3/5(Uref_Bn) -> [Uref_Bn_d]
  [Blk] -> Uref2m3/2(Block)
  Uref2m3/3(Uref_Cp) -> [Uref_Cp_d]
  Selector9/1 -> Selector12/1, Control2/4(Vsec)
  Uref2m3/1(Uref_Ap) -> [Uref_Ap_d]
  Control2/1(Uref) -> Uref2m3/1(Uref_ABC)
  [Qref] -> Control2/3(Qref)
  [PQreg_On] -> Control2/1(PQreg_ON)
  Uref2m3/2(Uref_Bp) -> [Uref_Bp_d]
  Mux59/1 -> Scope6/2
  Mux60/1 -> Scope6/1
  Selector10/1 -> Selector13/1
  [Vsec] -> Selector11/1
  [Idiode] -> Scope4/1, Demux17/1
  Selector11/1 -> Mux60/1  "EMT"
  Selector13/1 -> Mux60/2  "DQSYM"
  Selector14/1 -> Mux59/1  "EMT"
  Selector16/1 -> Mux59/2  "DQSYM"
  connections:
  Ld1/LConn1 -- RL Src/RConn1 -- prim/RConn1
  Ld1/LConn2 -- RL Src/RConn2 -- prim/RConn2
  Ld1/LConn3 -- RL Src/RConn3 -- prim/RConn3
  sec/RConn1 -- Ld2/LConn1 -- Tr1/RConn1
  sec/RConn2 -- Ld2/LConn2 -- Tr1/RConn2
  Ld2/LConn3 -- sec/RConn3 -- Tr1/RConn3
  R_startup/RConn1 -- Brk2/RConn1 -- Tr1/LConn1
  R_startup/RConn2 -- Brk2/RConn2 -- Tr1/LConn2
  R_startup/RConn3 -- Brk2/RConn3 -- Tr1/LConn3
  Voltage source/RConn3 -- RL Src/LConn3
  Voltage source/RConn2 -- RL Src/LConn2
  Voltage source/RConn1 -- RL Src/LConn1
  MMC/RConn1 -- DC & converter 2/LConn1 -- MMC1/RConn1
  MMC/LConn1 -- MMC1/LConn1 -- Voltage source1/RConn1 -- sec/LConn1
  MMC/RConn2 -- DC & converter 2/LConn2 -- MMC1/RConn2
  MMC/LConn2 -- MMC1/LConn2 -- Voltage source1/RConn2 -- sec/LConn2
  MMC/LConn3 -- MMC1/LConn3 -- Voltage source1/RConn3 -- sec/LConn3
  VS Conv2t/LConn1 -- VS Conv2b/RConn1 -- Ground2/LConn1
  Conv 2/LConn1 -- DC & converter 2/RConn1 -- VS Conv2t/RConn1
  Conv 2/LConn2 -- DC & converter 2/RConn2 -- VS Conv2b/LConn1
  Brk1/LConn1 -- prim/LConn1
  Brk1/LConn2 -- prim/LConn2
  Brk1/LConn3 -- prim/LConn3
  R_startup/LConn3 -- Brk2/LConn3 -- Brk1/RConn3
  Brk1/RConn2 -- Brk2/LConn2 -- R_startup/LConn2
  R_startup/LConn1 -- Brk2/LConn1 -- Brk1/RConn1
